simulink library "ammclib_bam_S32K3xx"  (R2016a)
(part 20 of 50)

      |     warning(['Parameter u16NShiftI of ' gcb ' exceeds the fixed-point range.']);
      |   end
      |   f32C1=round(c1f*2^(-u16NShiftI)*2^31);
      |   if f32C1>2^31-1
      |     f32C1=2^31-1;
      |     warning(['Parameter f32C1 of ' gcb ' exceeds the fixed-point range.']);
      |   end
      |   if f32C1<-2^31
      |     f32C1=-2^31;
      |     warning(['Parameter f32C1 of ' gcb ' exceeds the fixed-point range.']);
      |   end
      |   if isnan(f32CC1sc)
      |     if ~strcmp(f32CC1sc_bkup,'0')
      |       set_param(gcb,'f32CC1sc','0');
      |     end
      |   else
      |     tmps=num2str(f32CC1sc);
      |     if ~strcmp(f32CC1sc_bkup,tmps)
      |       set_param(gcb,'f32CC1sc',tmps);
      |     end
      |   end
      |   if isnan(f32CC2sc)
      |     if ~strcmp(f32CC2sc_bkup,'0')
      |       set_param(gcb,'f32CC2sc','0');
      |     end
      |   else
      |     tmps=num2str(f32CC2sc);
      |     if ~strcmp(f32CC2sc_bkup,tmps)
      |       set_param(gcb,'f32CC2sc',tmps);
      |     end
      |   end
      |   if isnan(f32UpperLimit)
      |     if ~strcmp(f32UpperLimit_bkup,'0')
      |       set_param(gcb,'f32UpperLimit','0');
      |     end
      |   else
      |     tmps=num2str(f32UpperLimit);
      |     if ~strcmp(f32UpperLimit_bkup,tmps)
      |       set_param(gcb,'f32UpperLimit',tmps);
      |     end
      |   end
      |   if isnan(f32LowerLimit)
      |     if ~strcmp(f32LowerLimit_bkup,'0')
      |       set_param(gcb,'f32LowerLimit','0');
      |     end
      |   else
      |     tmps=num2str(f32LowerLimit);
      |     if ~strcmp(f32LowerLimit_bkup,tmps)
      |       set_param(gcb,'f32LowerLimit',tmps);
      |     end
      |   end
      |   if isnan(u16NShiftPI)
      |     if ~strcmp(u16NShiftPI_bkup,'0')
      |       set_param(gcb,'u16NShiftPI','0');
      |     end
      |   else
      |     tmps=num2str(u16NShiftPI);
      |     if ~strcmp(u16NShiftPI_bkup,tmps)
      |       set_param(gcb,'u16NShiftPI',tmps);
      |     end
      |   end
      |   if isnan(f32C1)
      |     if ~strcmp(f32C1_bkup,'0')
      |       set_param(gcb,'f32C1','0');
      |     end
      |   else
      |     tmps=num2str(f32C1);
      |     if ~strcmp(f32C1_bkup,tmps)
      |       set_param(gcb,'f32C1',tmps);
      |     end
      |   end
      |   if isnan(u16NShiftI)
      |     if ~strcmp(u16NShiftI_bkup,'0')
      |       set_param(gcb,'u16NShiftI','0');
      |     end
      |   else
      |     tmps=num2str(u16NShiftI);
      |     if ~strcmp(u16NShiftI_bkup,tmps)
      |       set_param(gcb,'u16NShiftI',tmps);
      |     end
      |   end
      | end
      mask Callback if0:
      | autoCalcEn=get_param(gcb,'autoCalcEn');
      | if strcmp(autoCalcEn,'on')
      |   SampleTime=Simulink.data.evalinGlobal(bdroot,get_param(gcb,'SampleTime'));
      |   if (SampleTime==-1)
      |     SampleTime=str2double(get_param(gcb,'SampleTime_1'));
      |   end
      |   f32CC1sc_bkup=get_param(gcb,'f32CC1sc');
      |   f32CC2sc_bkup=get_param(gcb,'f32CC2sc');
      |   f32UpperLimit_bkup=get_param(gcb,'f32UpperLimit');
      |   f32LowerLimit_bkup=get_param(gcb,'f32LowerLimit');
      |   u16NShiftPI_bkup=get_param(gcb,'u16NShiftPI');
      |   f32C1_bkup=get_param(gcb,'f32C1');
      |   u16NShiftI_bkup=get_param(gcb,'u16NShiftI');
      |   intmethod=get_param(gcb,'intmethod');
      |   if0=Simulink.data.evalinGlobal(bdroot,get_param(gcb,'if0'));
      |   iksi=Simulink.data.evalinGlobal(bdroot,get_param(gcb,'iksi'));
      |   mechspeed=Simulink.data.evalinGlobal(bdroot,get_param(gcb,'mechspeed'));
      |   polepairs=Simulink.data.evalinGlobal(bdroot,get_param(gcb,'polepairs'));
      |   if (if0<=0)
      |     warning('Natural frequency f0 must be positive.');
      |   end
      |   if (iksi<=0)
      |     warning('Current loop attenuation must be positive.');
      |   end
      |   if (iksi>1)
      |     warning('Current loop attenuation must not exceed 1.');
      |   end
      |   if (mechspeed<=0)
      |     warning('Max. speed must be positive.');
      |   end
      |   if (polepairs<1)
      |     warning('Number of pole pairs must be a natural number (1, 2, 3, ...).');
      |   end
      |   if (round(polepairs)~=polepairs)
      |     warning('Number of pole pairs must be a natural number (1, 2, 3, ...).');
      |   end
      |   pgain=12.56637061435917*iksi*if0;
      |   igain=39.47841760435743*if0*if0;
      |   if strcmp(intmethod,'Forward Rectangular')
      |     cc1=pgain;
      |     cc2=-pgain+igain*SampleTime;
      |   else
      |     if strcmp(intmethod,'Backward Rectangular')
      |       cc1=pgain+igain*SampleTime;
      |       cc2=-pgain;
      |     else
      |       cc1=pgain+igain*SampleTime*0.5;
      |       cc2=-pgain+igain*SampleTime*0.5;
      |     end
      |   end
      |   wmax=polepairs*mechspeed*0.1047197551196598;
      |   cc1f=cc1*3.141592653589793/wmax;
      |   cc2f=cc2*3.141592653589793/wmax;
      |   u16NShiftPI=ceil(log2(abs(cc1f)));
      |   tmpsh=ceil(log2(abs(cc2f)));
      |   if u16NShiftPI<tmpsh
      |     u16NShiftPI=tmpsh;
      |   end
      |   if u16NShiftPI<0
      |     u16NShiftPI=0;
      |   end
      |   if u16NShiftPI>31
      |     u16NShiftPI=31;
      |     warning(['Parameter u16NShiftPI of ' gcb ' exceeds the fixed-point range.']);
      |   end
      |   f32CC1sc=round(cc1f*2^(-u16NShiftPI)*2^31);
      |   if f32CC1sc>2^31-1
      |     f32CC1sc=2^31-1;
      |     warning(['Parameter f32CC1sc of ' gcb ' exceeds the fixed-point range.']);
      |   end
      |   if f32CC1sc<-2^31
      |     f32CC1sc=-2^31;
      |     warning(['Parameter f32CC1sc of ' gcb ' exceeds the fixed-point range.']);
      |   end
      |   f32CC2sc=round(cc2f*2^(-u16NShiftPI)*2^31);
      |   if f32CC2sc>2^31-1
      |     f32CC2sc=2^31-1;
      |     warning(['Parameter f32CC2sc of ' gcb ' exceeds the fixed-point range.']);
      |   end
      |   if f32CC2sc<-2^31
      |     f32CC2sc=-2^31;
      |     warning(['Parameter f32CC2sc of ' gcb ' exceeds the fixed-point range.']);
      |   end
      |   f32LowerLimit=-2147483648;
      |   f32UpperLimit=2147483647;
      |   c1f=SampleTime*0.5*wmax/3.141592653589793;
      |   u16NShiftI=ceil(log2(abs(c1f)));
      |   if u16NShiftI<0
      |     u16NShiftI=0;
      |   end
      |   if u16NShiftI>31
      |     u16NShiftI=31;
      |     warning(['Parameter u16NShiftI of ' gcb ' exceeds the fixed-point range.']);
      |   end
      |   f32C1=round(c1f*2^(-u16NShiftI)*2^31);
      |   if f32C1>2^31-1
      |     f32C1=2^31-1;
      |     warning(['Parameter f32C1 of ' gcb ' exceeds the fixed-point range.']);
      |   end
      |   if f32C1<-2^31
      |     f32C1=-2^31;
      |     warning(['Parameter f32C1 of ' gcb ' exceeds the fixed-point range.']);
      |   end
      |   if isnan(f32CC1sc)
      |     if ~strcmp(f32CC1sc_bkup,'0')
      |       set_param(gcb,'f32CC1sc','0');
      |     end
      |   else
      |     tmps=num2str(f32CC1sc);
      |     if ~strcmp(f32CC1sc_bkup,tmps)
      |       set_param(gcb,'f32CC1sc',tmps);
      |     end
      |   end
      |   if isnan(f32CC2sc)
      |     if ~strcmp(f32CC2sc_bkup,'0')
      |       set_param(gcb,'f32CC2sc','0');
      |     end
      |   else
      |     tmps=num2str(f32CC2sc);
      |     if ~strcmp(f32CC2sc_bkup,tmps)
      |       set_param(gcb,'f32CC2sc',tmps);
      |     end
      |   end
      |   if isnan(f32UpperLimit)
      |     if ~strcmp(f32UpperLimit_bkup,'0')
      |       set_param(gcb,'f32UpperLimit','0');
      |     end
      |   else
      |     tmps=num2str(f32UpperLimit);
      |     if ~strcmp(f32UpperLimit_bkup,tmps)
      |       set_param(gcb,'f32UpperLimit',tmps);
      |     end
      |   end
      |   if isnan(f32LowerLimit)
      |     if ~strcmp(f32LowerLimit_bkup,'0')
      |       set_param(gcb,'f32LowerLimit','0');
      |     end
      |   else
      |     tmps=num2str(f32LowerLimit);
      |     if ~strcmp(f32LowerLimit_bkup,tmps)
      |       set_param(gcb,'f32LowerLimit',tmps);
      |     end
      |   end
      |   if isnan(u16NShiftPI)
      |     if ~strcmp(u16NShiftPI_bkup,'0')
      |       set_param(gcb,'u16NShiftPI','0');
      |     end
      |   else
      |     tmps=num2str(u16NShiftPI);
      |     if ~strcmp(u16NShiftPI_bkup,tmps)
      |       set_param(gcb,'u16NShiftPI',tmps);
      |     end
      |   end
      |   if isnan(f32C1)
      |     if ~strcmp(f32C1_bkup,'0')
      |       set_param(gcb,'f32C1','0');
      |     end
      |   else
      |     tmps=num2str(f32C1);
      |     if ~strcmp(f32C1_bkup,tmps)
      |       set_param(gcb,'f32C1',tmps);
      |     end
      |   end
      |   if isnan(u16NShiftI)
      |     if ~strcmp(u16NShiftI_bkup,'0')
      |       set_param(gcb,'u16NShiftI','0');
      |     end
      |   else
      |     tmps=num2str(u16NShiftI);
      |     if ~strcmp(u16NShiftI_bkup,tmps)
      |       set_param(gcb,'u16NShiftI',tmps);
      |     end
      |   end
      | end
      mask Callback iksi:
      | autoCalcEn=get_param(gcb,'autoCalcEn');
      | if strcmp(autoCalcEn,'on')
      |   SampleTime=Simulink.data.evalinGlobal(bdroot,get_param(gcb,'SampleTime'));
      |   if (SampleTime==-1)
      |     SampleTime=str2double(get_param(gcb,'SampleTime_1'));
      |   end
      |   f32CC1sc_bkup=get_param(gcb,'f32CC1sc');
      |   f32CC2sc_bkup=get_param(gcb,'f32CC2sc');
      |   f32UpperLimit_bkup=get_param(gcb,'f32UpperLimit');
      |   f32LowerLimit_bkup=get_param(gcb,'f32LowerLimit');
      |   u16NShiftPI_bkup=get_param(gcb,'u16NShiftPI');
      |   f32C1_bkup=get_param(gcb,'f32C1');
      |   u16NShiftI_bkup=get_param(gcb,'u16NShiftI');
      |   intmethod=get_param(gcb,'intmethod');
      |   if0=Simulink.data.evalinGlobal(bdroot,get_param(gcb,'if0'));
      |   iksi=Simulink.data.evalinGlobal(bdroot,get_param(gcb,'iksi'));
      |   mechspeed=Simulink.data.evalinGlobal(bdroot,get_param(gcb,'mechspeed'));
      |   polepairs=Simulink.data.evalinGlobal(bdroot,get_param(gcb,'polepairs'));
      |   if (if0<=0)
      |     warning('Natural frequency f0 must be positive.');
      |   end
      |   if (iksi<=0)
      |     warning('Current loop attenuation must be positive.');
      |   end
      |   if (iksi>1)
      |     warning('Current loop attenuation must not exceed 1.');
      |   end
      |   if (mechspeed<=0)
      |     warning('Max. speed must be positive.');
      |   end
      |   if (polepairs<1)
      |     warning('Number of pole pairs must be a natural number (1, 2, 3, ...).');
      |   end
      |   if (round(polepairs)~=polepairs)
      |     warning('Number of pole pairs must be a natural number (1, 2, 3, ...).');
      |   end
      |   pgain=12.56637061435917*iksi*if0;
      |   igain=39.47841760435743*if0*if0;
      |   if strcmp(intmethod,'Forward Rectangular')
      |     cc1=pgain;
      |     cc2=-pgain+igain*SampleTime;
      |   else
      |     if strcmp(intmethod,'Backward Rectangular')
      |       cc1=pgain+igain*SampleTime;
      |       cc2=-pgain;
      |     else
      |       cc1=pgain+igain*SampleTime*0.5;
      |       cc2=-pgain+igain*SampleTime*0.5;
      |     end
      |   end
      |   wmax=polepairs*mechspeed*0.1047197551196598;
      |   cc1f=cc1*3.141592653589793/wmax;
      |   cc2f=cc2*3.141592653589793/wmax;
      |   u16NShiftPI=ceil(log2(abs(cc1f)));
      |   tmpsh=ceil(log2(abs(cc2f)));
      |   if u16NShiftPI<tmpsh
      |     u16NShiftPI=tmpsh;
      |   end
      |   if u16NShiftPI<0
      |     u16NShiftPI=0;
      |   end
      |   if u16NShiftPI>31
      |     u16NShiftPI=31;
      |     warning(['Parameter u16NShiftPI of ' gcb ' exceeds the fixed-point range.']);
      |   end
      |   f32CC1sc=round(cc1f*2^(-u16NShiftPI)*2^31);
      |   if f32CC1sc>2^31-1
      |     f32CC1sc=2^31-1;
      |     warning(['Parameter f32CC1sc of ' gcb ' exceeds the fixed-point range.']);
      |   end
      |   if f32CC1sc<-2^31
      |     f32CC1sc=-2^31;
      |     warning(['Parameter f32CC1sc of ' gcb ' exceeds the fixed-point range.']);
      |   end
      |   f32CC2sc=round(cc2f*2^(-u16NShiftPI)*2^31);
      |   if f32CC2sc>2^31-1
      |     f32CC2sc=2^31-1;
      |     warning(['Parameter f32CC2sc of ' gcb ' exceeds the fixed-point range.']);
      |   end
      |   if f32CC2sc<-2^31
      |     f32CC2sc=-2^31;
      |     warning(['Parameter f32CC2sc of ' gcb ' exceeds the fixed-point range.']);
      |   end
      |   f32LowerLimit=-2147483648;
      |   f32UpperLimit=2147483647;
      |   c1f=SampleTime*0.5*wmax/3.141592653589793;
      |   u16NShiftI=ceil(log2(abs(c1f)));
      |   if u16NShiftI<0
      |     u16NShiftI=0;
      |   end
      |   if u16NShiftI>31
      |     u16NShiftI=31;
      |     warning(['Parameter u16NShiftI of ' gcb ' exceeds the fixed-point range.']);
      |   end
      |   f32C1=round(c1f*2^(-u16NShiftI)*2^31);
      |   if f32C1>2^31-1
      |     f32C1=2^31-1;
      |     warning(['Parameter f32C1 of ' gcb ' exceeds the fixed-point range.']);
      |   end
      |   if f32C1<-2^31
      |     f32C1=-2^31;
      |     warning(['Parameter f32C1 of ' gcb ' exceeds the fixed-point range.']);
      |   end
      |   if isnan(f32CC1sc)
      |     if ~strcmp(f32CC1sc_bkup,'0')
      |       set_param(gcb,'f32CC1sc','0');
      |     end
      |   else
      |     tmps=num2str(f32CC1sc);
      |     if ~strcmp(f32CC1sc_bkup,tmps)
      |       set_param(gcb,'f32CC1sc',tmps);
      |     end
      |   end
      |   if isnan(f32CC2sc)
      |     if ~strcmp(f32CC2sc_bkup,'0')
      |       set_param(gcb,'f32CC2sc','0');
      |     end
      |   else
      |     tmps=num2str(f32CC2sc);
      |     if ~strcmp(f32CC2sc_bkup,tmps)
      |       set_param(gcb,'f32CC2sc',tmps);
      |     end
      |   end
      |   if isnan(f32UpperLimit)
      |     if ~strcmp(f32UpperLimit_bkup,'0')
      |       set_param(gcb,'f32UpperLimit','0');
      |     end
      |   else
      |     tmps=num2str(f32UpperLimit);
      |     if ~strcmp(f32UpperLimit_bkup,tmps)
      |       set_param(gcb,'f32UpperLimit',tmps);
      |     end
      |   end
      |   if isnan(f32LowerLimit)
      |     if ~strcmp(f32LowerLimit_bkup,'0')
      |       set_param(gcb,'f32LowerLimit','0');
      |     end
      |   else
      |     tmps=num2str(f32LowerLimit);
      |     if ~strcmp(f32LowerLimit_bkup,tmps)
      |       set_param(gcb,'f32LowerLimit',tmps);
      |     end
      |   end
      |   if isnan(u16NShiftPI)
      |     if ~strcmp(u16NShiftPI_bkup,'0')
      |       set_param(gcb,'u16NShiftPI','0');
      |     end
      |   else
      |     tmps=num2str(u16NShiftPI);
      |     if ~strcmp(u16NShiftPI_bkup,tmps)
      |       set_param(gcb,'u16NShiftPI',tmps);
      |     end
      |   end
      |   if isnan(f32C1)
      |     if ~strcmp(f32C1_bkup,'0')
      |       set_param(gcb,'f32C1','0');
      |     end
      |   else
      |     tmps=num2str(f32C1);
      |     if ~strcmp(f32C1_bkup,tmps)
      |       set_param(gcb,'f32C1',tmps);
      |     end
      |   end
      |   if isnan(u16NShiftI)
      |     if ~strcmp(u16NShiftI_bkup,'0')
      |       set_param(gcb,'u16NShiftI','0');
      |     end
      |   else
      |     tmps=num2str(u16NShiftI);
      |     if ~strcmp(u16NShiftI_bkup,tmps)
      |       set_param(gcb,'u16NShiftI',tmps);
      |     end
      |   end
      | end
      mask Callback mechspeed:
      | autoCalcEn=get_param(gcb,'autoCalcEn');
      | if strcmp(autoCalcEn,'on')
      |   SampleTime=Simulink.data.evalinGlobal(bdroot,get_param(gcb,'SampleTime'));
      |   if (SampleTime==-1)
      |     SampleTime=str2double(get_param(gcb,'SampleTime_1'));
      |   end
      |   f32CC1sc_bkup=get_param(gcb,'f32CC1sc');
      |   f32CC2sc_bkup=get_param(gcb,'f32CC2sc');
      |   f32UpperLimit_bkup=get_param(gcb,'f32UpperLimit');
      |   f32LowerLimit_bkup=get_param(gcb,'f32LowerLimit');
      |   u16NShiftPI_bkup=get_param(gcb,'u16NShiftPI');
      |   f32C1_bkup=get_param(gcb,'f32C1');
      |   u16NShiftI_bkup=get_param(gcb,'u16NShiftI');
      |   intmethod=get_param(gcb,'intmethod');
      |   if0=Simulink.data.evalinGlobal(bdroot,get_param(gcb,'if0'));
      |   iksi=Simulink.data.evalinGlobal(bdroot,get_param(gcb,'iksi'));
      |   mechspeed=Simulink.data.evalinGlobal(bdroot,get_param(gcb,'mechspeed'));
      |   polepairs=Simulink.data.evalinGlobal(bdroot,get_param(gcb,'polepairs'));
      |   if (if0<=0)
      |     warning('Natural frequency f0 must be positive.');
      |   end
      |   if (iksi<=0)
      |     warning('Current loop attenuation must be positive.');
      |   end
      |   if (iksi>1)
      |     warning('Current loop attenuation must not exceed 1.');
      |   end
      |   if (mechspeed<=0)
      |     warning('Max. speed must be positive.');
      |   end
      |   if (polepairs<1)
      |     warning('Number of pole pairs must be a natural number (1, 2, 3, ...).');
      |   end
      |   if (round(polepairs)~=polepairs)
      |     warning('Number of pole pairs must be a natural number (1, 2, 3, ...).');
      |   end
      |   pgain=12.56637061435917*iksi*if0;
      |   igain=39.47841760435743*if0*if0;
      |   if strcmp(intmethod,'Forward Rectangular')
      |     cc1=pgain;
      |     cc2=-pgain+igain*SampleTime;
      |   else
      |     if strcmp(intmethod,'Backward Rectangular')
      |       cc1=pgain+igain*SampleTime;
      |       cc2=-pgain;
      |     else
      |       cc1=pgain+igain*SampleTime*0.5;
      |       cc2=-pgain+igain*SampleTime*0.5;
      |     end
      |   end
      |   wmax=polepairs*mechspeed*0.1047197551196598;
      |   cc1f=cc1*3.141592653589793/wmax;
      |   cc2f=cc2*3.141592653589793/wmax;
      |   u16NShiftPI=ceil(log2(abs(cc1f)));
      |   tmpsh=ceil(log2(abs(cc2f)));
      |   if u16NShiftPI<tmpsh
      |     u16NShiftPI=tmpsh;
      |   end
      |   if u16NShiftPI<0
      |     u16NShiftPI=0;
      |   end
      |   if u16NShiftPI>31
      |     u16NShiftPI=31;
      |     warning(['Parameter u16NShiftPI of ' gcb ' exceeds the fixed-point range.']);
      |   end
      |   f32CC1sc=round(cc1f*2^(-u16NShiftPI)*2^31);
      |   if f32CC1sc>2^31-1
      |     f32CC1sc=2^31-1;
      |     warning(['Parameter f32CC1sc of ' gcb ' exceeds the fixed-point range.']);
      |   end
      |   if f32CC1sc<-2^31
      |     f32CC1sc=-2^31;
      |     warning(['Parameter f32CC1sc of ' gcb ' exceeds the fixed-point range.']);
      |   end
      |   f32CC2sc=round(cc2f*2^(-u16NShiftPI)*2^31);
      |   if f32CC2sc>2^31-1
      |     f32CC2sc=2^31-1;
      |     warning(['Parameter f32CC2sc of ' gcb ' exceeds the fixed-point range.']);
      |   end
      |   if f32CC2sc<-2^31
      |     f32CC2sc=-2^31;
      |     warning(['Parameter f32CC2sc of ' gcb ' exceeds the fixed-point range.']);
      |   end
      |   f32LowerLimit=-2147483648;
      |   f32UpperLimit=2147483647;
      |   c1f=SampleTime*0.5*wmax/3.141592653589793;
      |   u16NShiftI=ceil(log2(abs(c1f)));
      |   if u16NShiftI<0
      |     u16NShiftI=0;
      |   end
      |   if u16NShiftI>31
      |     u16NShiftI=31;
      |     warning(['Parameter u16NShiftI of ' gcb ' exceeds the fixed-point range.']);
      |   end
      |   f32C1=round(c1f*2^(-u16NShiftI)*2^31);
      |   if f32C1>2^31-1
      |     f32C1=2^31-1;
      |     warning(['Parameter f32C1 of ' gcb ' exceeds the fixed-point range.']);
      |   end
      |   if f32C1<-2^31
      |     f32C1=-2^31;
      |     warning(['Parameter f32C1 of ' gcb ' exceeds the fixed-point range.']);
      |   end
      |   if isnan(f32CC1sc)
      |     if ~strcmp(f32CC1sc_bkup,'0')
      |       set_param(gcb,'f32CC1sc','0');
      |     end
      |   else
      |     tmps=num2str(f32CC1sc);
      |     if ~strcmp(f32CC1sc_bkup,tmps)
      |       set_param(gcb,'f32CC1sc',tmps);
      |     end
      |   end
      |   if isnan(f32CC2sc)
      |     if ~strcmp(f32CC2sc_bkup,'0')
      |       set_param(gcb,'f32CC2sc','0');
      |     end
      |   else
      |     tmps=num2str(f32CC2sc);
      |     if ~strcmp(f32CC2sc_bkup,tmps)
      |       set_param(gcb,'f32CC2sc',tmps);
      |     end
      |   end
      |   if isnan(f32UpperLimit)
      |     if ~strcmp(f32UpperLimit_bkup,'0')
      |       set_param(gcb,'f32UpperLimit','0');
      |     end
      |   else
      |     tmps=num2str(f32UpperLimit);
      |     if ~strcmp(f32UpperLimit_bkup,tmps)
      |       set_param(gcb,'f32UpperLimit',tmps);
      |     end
      |   end
      |   if isnan(f32LowerLimit)
      |     if ~strcmp(f32LowerLimit_bkup,'0')
      |       set_param(gcb,'f32LowerLimit','0');
      |     end
      |   else
      |     tmps=num2str(f32LowerLimit);
      |     if ~strcmp(f32LowerLimit_bkup,tmps)
      |       set_param(gcb,'f32LowerLimit',tmps);
      |     end
      |   end
      |   if isnan(u16NShiftPI)
      |     if ~strcmp(u16NShiftPI_bkup,'0')
      |       set_param(gcb,'u16NShiftPI','0');
      |     end
      |   else
      |     tmps=num2str(u16NShiftPI);
      |     if ~strcmp(u16NShiftPI_bkup,tmps)
      |       set_param(gcb,'u16NShiftPI',tmps);
      |     end
      |   end
      |   if isnan(f32C1)
      |     if ~strcmp(f32C1_bkup,'0')
      |       set_param(gcb,'f32C1','0');
      |     end
      |   else
      |     tmps=num2str(f32C1);
      |     if ~strcmp(f32C1_bkup,tmps)
      |       set_param(gcb,'f32C1',tmps);
      |     end
      |   end
      |   if isnan(u16NShiftI)
      |     if ~strcmp(u16NShiftI_bkup,'0')
      |       set_param(gcb,'u16NShiftI','0');
      |     end
      |   else
      |     tmps=num2str(u16NShiftI);
      |     if ~strcmp(u16NShiftI_bkup,tmps)
      |       set_param(gcb,'u16NShiftI',tmps);
      |     end
      |   end
      | end
      mask Callback polepairs:
      | autoCalcEn=get_param(gcb,'autoCalcEn');
      | if strcmp(autoCalcEn,'on')
      |   SampleTime=Simulink.data.evalinGlobal(bdroot,get_param(gcb,'SampleTime'));
      |   if (SampleTime==-1)
      |     SampleTime=str2double(get_param(gcb,'SampleTime_1'));
      |   end
      |   f32CC1sc_bkup=get_param(gcb,'f32CC1sc');
      |   f32CC2sc_bkup=get_param(gcb,'f32CC2sc');
      |   f32UpperLimit_bkup=get_param(gcb,'f32UpperLimit');
      |   f32LowerLimit_bkup=get_param(gcb,'f32LowerLimit');
      |   u16NShiftPI_bkup=get_param(gcb,'u16NShiftPI');
      |   f32C1_bkup=get_param(gcb,'f32C1');
      |   u16NShiftI_bkup=get_param(gcb,'u16NShiftI');
      |   intmethod=get_param(gcb,'intmethod');
      |   if0=Simulink.data.evalinGlobal(bdroot,get_param(gcb,'if0'));
      |   iksi=Simulink.data.evalinGlobal(bdroot,get_param(gcb,'iksi'));
      |   mechspeed=Simulink.data.evalinGlobal(bdroot,get_param(gcb,'mechspeed'));
      |   polepairs=Simulink.data.evalinGlobal(bdroot,get_param(gcb,'polepairs'));
      |   if (if0<=0)
      |     warning('Natural frequency f0 must be positive.');
      |   end
      |   if (iksi<=0)
      |     warning('Current loop attenuation must be positive.');
      |   end
      |   if (iksi>1)
      |     warning('Current loop attenuation must not exceed 1.');
      |   end
      |   if (mechspeed<=0)
      |     warning('Max. speed must be positive.');
      |   end
      |   if (polepairs<1)
      |     warning('Number of pole pairs must be a natural number (1, 2, 3, ...).');
      |   end
      |   if (round(polepairs)~=polepairs)
      |     warning('Number of pole pairs must be a natural number (1, 2, 3, ...).');
      |   end
      |   pgain=12.56637061435917*iksi*if0;
      |   igain=39.47841760435743*if0*if0;
      |   if strcmp(intmethod,'Forward Rectangular')
      |     cc1=pgain;
      |     cc2=-pgain+igain*SampleTime;
      |   else
      |     if strcmp(intmethod,'Backward Rectangular')
      |       cc1=pgain+igain*SampleTime;
      |       cc2=-pgain;
      |     else
      |       cc1=pgain+igain*SampleTime*0.5;
      |       cc2=-pgain+igain*SampleTime*0.5;
      |     end
      |   end
      |   wmax=polepairs*mechspeed*0.1047197551196598;
      |   cc1f=cc1*3.141592653589793/wmax;
      |   cc2f=cc2*3.141592653589793/wmax;
      |   u16NShiftPI=ceil(log2(abs(cc1f)));
      |   tmpsh=ceil(log2(abs(cc2f)));
      |   if u16NShiftPI<tmpsh
      |     u16NShiftPI=tmpsh;
      |   end
      |   if u16NShiftPI<0
      |     u16NShiftPI=0;
      |   end
      |   if u16NShiftPI>31
      |     u16NShiftPI=31;
      |     warning(['Parameter u16NShiftPI of ' gcb ' exceeds the fixed-point range.']);
      |   end
      |   f32CC1sc=round(cc1f*2^(-u16NShiftPI)*2^31);
      |   if f32CC1sc>2^31-1
      |     f32CC1sc=2^31-1;
      |     warning(['Parameter f32CC1sc of ' gcb ' exceeds the fixed-point range.']);
      |   end
      |   if f32CC1sc<-2^31
      |     f32CC1sc=-2^31;
      |     warning(['Parameter f32CC1sc of ' gcb ' exceeds the fixed-point range.']);
      |   end
      |   f32CC2sc=round(cc2f*2^(-u16NShiftPI)*2^31);
      |   if f32CC2sc>2^31-1
      |     f32CC2sc=2^31-1;
      |     warning(['Parameter f32CC2sc of ' gcb ' exceeds the fixed-point range.']);
      |   end
      |   if f32CC2sc<-2^31
      |     f32CC2sc=-2^31;
      |     warning(['Parameter f32CC2sc of ' gcb ' exceeds the fixed-point range.']);
      |   end
      |   f32LowerLimit=-2147483648;
      |   f32UpperLimit=2147483647;
      |   c1f=SampleTime*0.5*wmax/3.141592653589793;
      |   u16NShiftI=ceil(log2(abs(c1f)));
      |   if u16NShiftI<0
      |     u16NShiftI=0;
      |   end
      |   if u16NShiftI>31
      |     u16NShiftI=31;
      |     warning(['Parameter u16NShiftI of ' gcb ' exceeds the fixed-point range.']);
      |   end
      |   f32C1=round(c1f*2^(-u16NShiftI)*2^31);
      |   if f32C1>2^31-1
      |     f32C1=2^31-1;
      |     warning(['Parameter f32C1 of ' gcb ' exceeds the fixed-point range.']);
      |   end
      |   if f32C1<-2^31
      |     f32C1=-2^31;
      |     warning(['Parameter f32C1 of ' gcb ' exceeds the fixed-point range.']);
      |   end
      |   if isnan(f32CC1sc)
      |     if ~strcmp(f32CC1sc_bkup,'0')
      |       set_param(gcb,'f32CC1sc','0');
      |     end
      |   else
      |     tmps=num2str(f32CC1sc);
      |     if ~strcmp(f32CC1sc_bkup,tmps)
      |       set_param(gcb,'f32CC1sc',tmps);
      |     end
      |   end
      |   if isnan(f32CC2sc)
      |     if ~strcmp(f32CC2sc_bkup,'0')
      |       set_param(gcb,'f32CC2sc','0');
      |     end
      |   else
      |     tmps=num2str(f32CC2sc);
      |     if ~strcmp(f32CC2sc_bkup,tmps)
      |       set_param(gcb,'f32CC2sc',tmps);
      |     end
      |   end
      |   if isnan(f32UpperLimit)
      |     if ~strcmp(f32UpperLimit_bkup,'0')
      |       set_param(gcb,'f32UpperLimit','0');
      |     end
      |   else
      |     tmps=num2str(f32UpperLimit);
      |     if ~strcmp(f32UpperLimit_bkup,tmps)
      |       set_param(gcb,'f32UpperLimit',tmps);
      |     end
      |   end
      |   if isnan(f32LowerLimit)
      |     if ~strcmp(f32LowerLimit_bkup,'0')
      |       set_param(gcb,'f32LowerLimit','0');
      |     end
      |   else
      |     tmps=num2str(f32LowerLimit);
      |     if ~strcmp(f32LowerLimit_bkup,tmps)
      |       set_param(gcb,'f32LowerLimit',tmps);
      |     end
      |   end
      |   if isnan(u16NShiftPI)
      |     if ~strcmp(u16NShiftPI_bkup,'0')
      |       set_param(gcb,'u16NShiftPI','0');
      |     end
      |   else
      |     tmps=num2str(u16NShiftPI);
      |     if ~strcmp(u16NShiftPI_bkup,tmps)
      |       set_param(gcb,'u16NShiftPI',tmps);
      |     end
      |   end
      |   if isnan(f32C1)
      |     if ~strcmp(f32C1_bkup,'0')
      |       set_param(gcb,'f32C1','0');
      |     end
      |   else
      |     tmps=num2str(f32C1);
      |     if ~strcmp(f32C1_bkup,tmps)
      |       set_param(gcb,'f32C1',tmps);
      |     end
      |   end
      |   if isnan(u16NShiftI)
      |     if ~strcmp(u16NShiftI_bkup,'0')
      |       set_param(gcb,'u16NShiftI','0');
      |     end
      |   else
      |     tmps=num2str(u16NShiftI);
      |     if ~strcmp(u16NShiftI_bkup,tmps)
      |       set_param(gcb,'u16NShiftI',tmps);
      |     end
      |   end
      | end
      mask Callback autoCalcEn:
      | maskStr=get_param(gcb,'showStates');
      | if strcmp(maskStr,'Hide (faster execution)')
      |   p=Simulink.Mask.get(gcb);
      |   autoCalcEn=get_param(gcb,'autoCalcEn');
      |   hintText=p.getDialogControl('timeHint');
      |   if strcmp(autoCalcEn,'on')
      |     param=p.getParameter('polepairs');
      |     if strcmp(param.Enabled,'off')
      |       SampleTime=Simulink.data.evalinGlobal(bdroot,get_param(gcb,'SampleTime'));
      |       if SampleTime==-1
      |         SampleTime=str2double(get_param(gcb,'SampleTime_1'));
      |         if isnan(SampleTime)
      |           hintText.Prompt=['Note: Implementation parameters cannot be calculated yet because the block''s inherited sample time is unknown. Simulink will update the sample time when you run the simulation.'];
      |         else
      |           hintText.Prompt=['Caution: Implementation parameters depend on inherited sample time. Make sure that the sample time of the block''s inputs corresponds to the sampling period in the target application.'];
      |         end
      |       else
      |         hintText.Prompt='Caution: Implementation parameters depend on the sample time. Make sure that the simulation time step corresponds to the sampling period in the target application.';
      |       end
      |       p=Simulink.Mask.get(gcb);
      |       param=p.getParameter('intmethod');
      |       param.set('Enabled','on');
      |       param=p.getParameter('if0');
      |       param.set('Enabled','on');
      |       param=p.getParameter('iksi');
      |       param.set('Enabled','on');
      |       param=p.getParameter('mechspeed');
      |       param.set('Enabled','on');
      |       param=p.getParameter('polepairs');
      |       param.set('Enabled','on');
      |     else
      |       SampleTime=Simulink.data.evalinGlobal(bdroot,get_param(gcb,'SampleTime'));
      |       if SampleTime==-1
      |         SampleTime=str2double(get_param(gcb,'SampleTime_1'));
      |       end
      |     end
      |     f32CC1sc_bkup=get_param(gcb,'f32CC1sc');
      |     f32CC2sc_bkup=get_param(gcb,'f32CC2sc');
      |     f32UpperLimit_bkup=get_param(gcb,'f32UpperLimit');
      |     f32LowerLimit_bkup=get_param(gcb,'f32LowerLimit');
      |     u16NShiftPI_bkup=get_param(gcb,'u16NShiftPI');
      |     f32C1_bkup=get_param(gcb,'f32C1');
      |     u16NShiftI_bkup=get_param(gcb,'u16NShiftI');
      |     intmethod=get_param(gcb,'intmethod');
      |     if0=Simulink.data.evalinGlobal(bdroot,get_param(gcb,'if0'));
      |     iksi=Simulink.data.evalinGlobal(bdroot,get_param(gcb,'iksi'));
      |     mechspeed=Simulink.data.evalinGlobal(bdroot,get_param(gcb,'mechspeed'));
      |     polepairs=Simulink.data.evalinGlobal(bdroot,get_param(gcb,'polepairs'));
      |     if (if0<=0)
      |       warning('Natural frequency f0 must be positive.');
      |     end
      |     if (iksi<=0)
      |       warning('Current loop attenuation must be positive.');
      |     end
      |     if (iksi>1)
      |       warning('Current loop attenuation must not exceed 1.');
      |     end
      |     if (mechspeed<=0)
      |       warning('Max. speed must be positive.');
      |     end
      |     if (polepairs<1)
      |       warning('Number of pole pairs must be a natural number (1, 2, 3, ...).');
      |     end
      |     if (round(polepairs)~=polepairs)
      |       warning('Number of pole pairs must be a natural number (1, 2, 3, ...).');
      |     end
      |     pgain=12.56637061435917*iksi*if0;
      |     igain=39.47841760435743*if0*if0;
      |     if strcmp(intmethod,'Forward Rectangular')
      |       cc1=pgain;
      |       cc2=-pgain+igain*SampleTime;
      |     else
      |       if strcmp(intmethod,'Backward Rectangular')
      |         cc1=pgain+igain*SampleTime;
      |         cc2=-pgain;
      |       else
      |         cc1=pgain+igain*SampleTime*0.5;
      |         cc2=-pgain+igain*SampleTime*0.5;
      |       end
      |     end
      |     wmax=polepairs*mechspeed*0.1047197551196598;
      |     cc1f=cc1*3.141592653589793/wmax;
      |     cc2f=cc2*3.141592653589793/wmax;
      |     u16NShiftPI=ceil(log2(abs(cc1f)));
      |     tmpsh=ceil(log2(abs(cc2f)));
      |     if u16NShiftPI<tmpsh
      |       u16NShiftPI=tmpsh;
      |     end
      |     if u16NShiftPI<0
      |       u16NShiftPI=0;
      |     end
      |     if u16NShiftPI>31
      |       u16NShiftPI=31;
      |       warning(['Parameter u16NShiftPI of ' gcb ' exceeds the fixed-point range.']);
      |     end
      |     f32CC1sc=round(cc1f*2^(-u16NShiftPI)*2^31);
      |     if f32CC1sc>2^31-1
      |       f32CC1sc=2^31-1;
      |       warning(['Parameter f32CC1sc of ' gcb ' exceeds the fixed-point range.']);
      |     end
      |     if f32CC1sc<-2^31
      |       f32CC1sc=-2^31;
      |       warning(['Parameter f32CC1sc of ' gcb ' exceeds the fixed-point range.']);
      |     end
      |     f32CC2sc=round(cc2f*2^(-u16NShiftPI)*2^31);
      |     if f32CC2sc>2^31-1
      |       f32CC2sc=2^31-1;
      |       warning(['Parameter f32CC2sc of ' gcb ' exceeds the fixed-point range.']);
      |     end
      |     if f32CC2sc<-2^31
      |       f32CC2sc=-2^31;
      |       warning(['Parameter f32CC2sc of ' gcb ' exceeds the fixed-point range.']);
      |     end
      |     f32LowerLimit=-2147483648;
      |     f32UpperLimit=2147483647;
      |     c1f=SampleTime*0.5*wmax/3.141592653589793;
      |     u16NShiftI=ceil(log2(abs(c1f)));
      |     if u16NShiftI<0
      |       u16NShiftI=0;
      |     end
      |     if u16NShiftI>31
      |       u16NShiftI=31;
      |       warning(['Parameter u16NShiftI of ' gcb ' exceeds the fixed-point range.']);
      |     end
      |     f32C1=round(c1f*2^(-u16NShiftI)*2^31);
      |     if f32C1>2^31-1
      |       f32C1=2^31-1;
      |       warning(['Parameter f32C1 of ' gcb ' exceeds the fixed-point range.']);
      |     end
      |     if f32C1<-2^31
      |       f32C1=-2^31;
      |       warning(['Parameter f32C1 of ' gcb ' exceeds the fixed-point range.']);
      |     end
      |     if isnan(f32CC1sc)
      |       if ~strcmp(f32CC1sc_bkup,'0')
      |         set_param(gcb,'f32CC1sc','0');
      |       end
      |     else
      |       tmps=num2str(f32CC1sc);
      |       if ~strcmp(f32CC1sc_bkup,tmps)
      |         set_param(gcb,'f32CC1sc',tmps);
      |       end
      |     end
      |     if isnan(f32CC2sc)
      |       if ~strcmp(f32CC2sc_bkup,'0')
      |         set_param(gcb,'f32CC2sc','0');
      |       end
      |     else
      |       tmps=num2str(f32CC2sc);
      |       if ~strcmp(f32CC2sc_bkup,tmps)
      |         set_param(gcb,'f32CC2sc',tmps);
      |       end
      |     end
      |     if isnan(f32UpperLimit)
      |       if ~strcmp(f32UpperLimit_bkup,'0')
      |         set_param(gcb,'f32UpperLimit','0');
      |       end
      |     else
      |       tmps=num2str(f32UpperLimit);
      |       if ~strcmp(f32UpperLimit_bkup,tmps)
      |         set_param(gcb,'f32UpperLimit',tmps);
      |       end
      |     end
      |     if isnan(f32LowerLimit)
      |       if ~strcmp(f32LowerLimit_bkup,'0')
      |         set_param(gcb,'f32LowerLimit','0');
      |       end
      |     else
      |       tmps=num2str(f32LowerLimit);
      |       if ~strcmp(f32LowerLimit_bkup,tmps)
      |         set_param(gcb,'f32LowerLimit',tmps);
      |       end
      |     end
      |     if isnan(u16NShiftPI)
      |       if ~strcmp(u16NShiftPI_bkup,'0')
      |         set_param(gcb,'u16NShiftPI','0');
      |       end
      |     else
      |       tmps=num2str(u16NShiftPI);
      |       if ~strcmp(u16NShiftPI_bkup,tmps)
      |         set_param(gcb,'u16NShiftPI',tmps);
      |       end
      |     end
      |     if isnan(f32C1)
      |       if ~strcmp(f32C1_bkup,'0')
      |         set_param(gcb,'f32C1','0');
      |       end
      |     else
      |       tmps=num2str(f32C1);
      |       if ~strcmp(f32C1_bkup,tmps)
      |         set_param(gcb,'f32C1',tmps);
      |       end
      |     end
      |     if isnan(u16NShiftI)
      |       if ~strcmp(u16NShiftI_bkup,'0')
      |         set_param(gcb,'u16NShiftI','0');
      |       end
      |     else
      |       tmps=num2str(u16NShiftI);
      |       if ~strcmp(u16NShiftI_bkup,tmps)
      |         set_param(gcb,'u16NShiftI',tmps);
      |       end
      |     end
      |   else
      |     param=p.getParameter('polepairs');
      |     if strcmp(param.Enabled,'on')
      |       hintText.Prompt='Caution: Implementation parameters are fixed.';
      |       p=Simulink.Mask.get(gcb);
      |       param=p.getParameter('intmethod');
      |       param.set('Enabled','off');
      |       param=p.getParameter('if0');
      |       param.set('Enabled','off');
      |       param=p.getParameter('iksi');
      |       param.set('Enabled','off');
      |       param=p.getParameter('mechspeed');
      |       param.set('Enabled','off');
      |       param=p.getParameter('polepairs');
      |       param.set('Enabled','off');
      |     end
      |   end
      | end
      mask DialogControl CompBut Prompt: Recalculate sample times
      mask DialogControl CompBut Tooltip: Simulink updates the sample times of all blocks when the simulation is run. This button will update the sample times now.
      mask DialogControl CompBut Callback:
      | btn=questdlg('This will apply all changes in all open dialog boxes and update the schematic. Do you want to proceed?','Apply all changes','Continue','Cancel','Continue');
      | if strcmp(btn,'Continue')
      |   dlgs=DAStudio.ToolRoot.getOpenDialogs;
      |   for i=1:length(dlgs)
      |     dlgs(i).apply;
      |   end
      |   try
      |     SampleTime_1=str2double(get_param(gcb,'SampleTime_1'));
      |     ts=Simulink.Block.getSampleTimes(gcb);
      |     ts=ts(1).Value(1);
      |     if (SampleTime_1 ~= ts)
      |       SampleTime_1=ts;
      |       set_param(gcb,'SampleTime_1',num2str(ts));
      |       autoCalcEn=get_param(gcb,'autoCalcEn');
      |       if strcmp(autoCalcEn,'on')
      |         SampleTime=Simulink.data.evalinGlobal(bdroot,get_param(gcb,'SampleTime'));
      |         p=Simulink.Mask.get(gcb);
      |         hintText=p.getDialogControl('timeHint');
      |         if SampleTime==-1
      |           SampleTime=SampleTime_1;
      |           hintText.Prompt='Caution: Implementation parameters depend on inherited sample time. Make sure that the sample time of the block''s inputs corresponds to the sampling period in the target application.';
      |         else
      |           hintText.Prompt='Caution: Implementation parameters depend on the sample time. Make sure that the simulation time step corresponds to the sampling period in the target application.';
      |         end
      |         f32CC1sc_bkup=get_param(gcb,'f32CC1sc');
      |         f32CC2sc_bkup=get_param(gcb,'f32CC2sc');
      |         f32UpperLimit_bkup=get_param(gcb,'f32UpperLimit');
      |         f32LowerLimit_bkup=get_param(gcb,'f32LowerLimit');
      |         u16NShiftPI_bkup=get_param(gcb,'u16NShiftPI');
      |         f32C1_bkup=get_param(gcb,'f32C1');
      |         u16NShiftI_bkup=get_param(gcb,'u16NShiftI');
      |         intmethod=get_param(gcb,'intmethod');
      |         if0=Simulink.data.evalinGlobal(bdroot,get_param(gcb,'if0'));
      |         iksi=Simulink.data.evalinGlobal(bdroot,get_param(gcb,'iksi'));
      |         mechspeed=Simulink.data.evalinGlobal(bdroot,get_param(gcb,'mechspeed'));
      |         polepairs=Simulink.data.evalinGlobal(bdroot,get_param(gcb,'polepairs'));
      |         if (if0<=0)
      |           warning('Natural frequency f0 must be positive.');
      |         end
      |         if (iksi<=0)
      |           warning('Current loop attenuation must be positive.');
      |         end
      |         if (iksi>1)
      |           warning('Current loop attenuation must not exceed 1.');
      |         end
      |         if (mechspeed<=0)
      |           warning('Max. speed must be positive.');
      |         end
      |         if (polepairs<1)
      |           warning('Number of pole pairs must be a natural number (1, 2, 3, ...).');
      |         end
      |         if (round(polepairs)~=polepairs)
      |           warning('Number of pole pairs must be a natural number (1, 2, 3, ...).');
      |         end
      |         pgain=12.56637061435917*iksi*if0;
      |         igain=39.47841760435743*if0*if0;
      |         if strcmp(intmethod,'Forward Rectangular')
      |           cc1=pgain;
      |           cc2=-pgain+igain*SampleTime;
      |         else
      |           if strcmp(intmethod,'Backward Rectangular')
      |             cc1=pgain+igain*SampleTime;
      |             cc2=-pgain;
      |           else
      |             cc1=pgain+igain*SampleTime*0.5;
      |             cc2=-pgain+igain*SampleTime*0.5;
      |           end
      |         end
      |         wmax=polepairs*mechspeed*0.1047197551196598;
      |         cc1f=cc1*3.141592653589793/wmax;
      |         cc2f=cc2*3.141592653589793/wmax;
      |         u16NShiftPI=ceil(log2(abs(cc1f)));
      |         tmpsh=ceil(log2(abs(cc2f)));
      |         if u16NShiftPI<tmpsh
      |           u16NShiftPI=tmpsh;
      |         end
      |         if u16NShiftPI<0
      |           u16NShiftPI=0;
      |         end
      |         if u16NShiftPI>31
      |           u16NShiftPI=31;
      |           warning(['Parameter u16NShiftPI of ' gcb ' exceeds the fixed-point range.']);
      |         end
      |         f32CC1sc=round(cc1f*2^(-u16NShiftPI)*2^31);
      |         if f32CC1sc>2^31-1
      |           f32CC1sc=2^31-1;
      |           warning(['Parameter f32CC1sc of ' gcb ' exceeds the fixed-point range.']);
      |         end
      |         if f32CC1sc<-2^31
      |           f32CC1sc=-2^31;
      |           warning(['Parameter f32CC1sc of ' gcb ' exceeds the fixed-point range.']);
      |         end
      |         f32CC2sc=round(cc2f*2^(-u16NShiftPI)*2^31);
      |         if f32CC2sc>2^31-1
      |           f32CC2sc=2^31-1;
      |           warning(['Parameter f32CC2sc of ' gcb ' exceeds the fixed-point range.']);
      |         end
      |         if f32CC2sc<-2^31
      |           f32CC2sc=-2^31;
      |           warning(['Parameter f32CC2sc of ' gcb ' exceeds the fixed-point range.']);
      |         end
      |         f32LowerLimit=-2147483648;
      |         f32UpperLimit=2147483647;
      |         c1f=SampleTime*0.5*wmax/3.141592653589793;
      |         u16NShiftI=ceil(log2(abs(c1f)));
      |         if u16NShiftI<0
      |           u16NShiftI=0;
      |         end
      |         if u16NShiftI>31
      |           u16NShiftI=31;
      |           warning(['Parameter u16NShiftI of ' gcb ' exceeds the fixed-point range.']);
      |         end
      |         f32C1=round(c1f*2^(-u16NShiftI)*2^31);
      |         if f32C1>2^31-1
      |           f32C1=2^31-1;
      |           warning(['Parameter f32C1 of ' gcb ' exceeds the fixed-point range.']);
      |         end
      |         if f32C1<-2^31
      |           f32C1=-2^31;
      |           warning(['Parameter f32C1 of ' gcb ' exceeds the fixed-point range.']);
      |         end
      |         if isnan(f32CC1sc)
      |           if ~strcmp(f32CC1sc_bkup,'0')
      |             set_param(gcb,'f32CC1sc','0');
      |           end
      |         else
      |           tmps=num2str(f32CC1sc);
      |           if ~strcmp(f32CC1sc_bkup,tmps)
      |             set_param(gcb,'f32CC1sc',tmps);
      |           end
      |         end
      |         if isnan(f32CC2sc)
      |           if ~strcmp(f32CC2sc_bkup,'0')
      |             set_param(gcb,'f32CC2sc','0');
      |           end
      |         else
      |           tmps=num2str(f32CC2sc);
      |           if ~strcmp(f32CC2sc_bkup,tmps)
      |             set_param(gcb,'f32CC2sc',tmps);
      |           end
      |         end
      |         if isnan(f32UpperLimit)
      |           if ~strcmp(f32UpperLimit_bkup,'0')
      |             set_param(gcb,'f32UpperLimit','0');
      |           end
      |         else
      |           tmps=num2str(f32UpperLimit);
      |           if ~strcmp(f32UpperLimit_bkup,tmps)
      |             set_param(gcb,'f32UpperLimit',tmps);
      |           end
      |         end
      |         if isnan(f32LowerLimit)
      |           if ~strcmp(f32LowerLimit_bkup,'0')
      |             set_param(gcb,'f32LowerLimit','0');
      |           end
      |         else
      |           tmps=num2str(f32LowerLimit);
      |           if ~strcmp(f32LowerLimit_bkup,tmps)
      |             set_param(gcb,'f32LowerLimit',tmps);
      |           end
      |         end
      |         if isnan(u16NShiftPI)
      |           if ~strcmp(u16NShiftPI_bkup,'0')
      |             set_param(gcb,'u16NShiftPI','0');
      |           end
      |         else
      |           tmps=num2str(u16NShiftPI);
      |           if ~strcmp(u16NShiftPI_bkup,tmps)
      |             set_param(gcb,'u16NShiftPI',tmps);
      |           end
      |         end
      |         if isnan(f32C1)
      |           if ~strcmp(f32C1_bkup,'0')
      |             set_param(gcb,'f32C1','0');
      |           end
      |         else
      |           tmps=num2str(f32C1);
      |           if ~strcmp(f32C1_bkup,tmps)
      |             set_param(gcb,'f32C1',tmps);
      |           end
      |         end
      |         if isnan(u16NShiftI)
      |           if ~strcmp(u16NShiftI_bkup,'0')
      |             set_param(gcb,'u16NShiftI','0');
      |           end
      |         else
      |           tmps=num2str(u16NShiftI);
      |           if ~strcmp(u16NShiftI_bkup,tmps)
      |             set_param(gcb,'u16NShiftI',tmps);
      |           end
      |         end
      |       end
      |     end
      |   catch
      |    warning(['Sample time cannot be calculated for the block ' gcb])
      |   end
      | end
      mask DialogControl timeHint Prompt: Note: Implementation parameters cannot be calculated yet because the block's inherited sample time is unknown. Simulink will update the sample time when you run the simulation.
      mask Display:
      | color('black');
      | pos = get_param(gcb, 'Position');
      | width = pos(3) - pos(1);
      | height = pos(4) - pos(2);
      | tX=width/2;
      | tY=height - 25;
      | color('black');
      | text(tX,tY, 'AMCLIB_TrackObsrv_F32', 'horizontalAlignment', 'center');
      | if showStates == 2
      |   color('red');
      |   text(tX,tY - 20, ['debugging mode' char(13) char(10) '(limited performance)'], 'horizontalAlignment', 'center');
      | end
  AMCLIB_Windmilling_F32 : Subsystem  StartFcn=|  TreatAsAtomicUnit=on  mask(AMCLIB_Windmilling_F32){showStates=Hide (faster execution), SampleTime=-1, if0=350, iksi=1, mechspeed=3000, polepairs=1, ADCMaxError=0.002, uscale=12, autoCalcEn=on, f32ADCMaxError=0, f32CC1sc=0, f32CC2sc=0, f32UpperLimit=0, f32LowerLimit=0, u16NShiftPI=0, f32C1=0, u16NShiftI=0, SampleTime_1=NaN}
      | ts=get_param(gcb,'CompiledSampleTime');
      | if iscell(ts)
      |   ts=ts{1};
      |   if iscell(ts)
      |     ts=ts{1};
      |   end
      | end
      | ts=ts(1);
      | set_param(gcb,'SampleTime_1',num2str(ts));
      | p=Simulink.Mask.get(gcb);
      | hintText=p.getDialogControl('timeHint');
      | SampleTime=Simulink.data.evalinGlobal(bdroot,get_param(gcb,'SampleTime'));
      | p=Simulink.Mask.get(gcb);
      | autoCalcEn=get_param(gcb,'autoCalcEn');
      | if strcmp(autoCalcEn,'on')
      |   if SampleTime==-1
      |     hintText.Prompt='Caution: Implementation parameters depend on inherited sample time. Make sure that the sample time of the block''s inputs corresponds to the sampling period in the target application.';
      |   else
      |     hintText.Prompt='Caution: Implementation parameters depend on the sample time. Make sure that the simulation time step corresponds to the sampling period in the target application.';
      |   end
      |   SampleTime=ts;
      |   f32ADCMaxError_bkup=get_param(gcb,'f32ADCMaxError');
      |   f32CC1sc_bkup=get_param(gcb,'f32CC1sc');
      |   f32CC2sc_bkup=get_param(gcb,'f32CC2sc');
      |   f32UpperLimit_bkup=get_param(gcb,'f32UpperLimit');
      |   f32LowerLimit_bkup=get_param(gcb,'f32LowerLimit');
      |   u16NShiftPI_bkup=get_param(gcb,'u16NShiftPI');
      |   f32C1_bkup=get_param(gcb,'f32C1');
      |   u16NShiftI_bkup=get_param(gcb,'u16NShiftI');
      |   if0=Simulink.data.evalinGlobal(bdroot,get_param(gcb,'if0'));
      |   iksi=Simulink.data.evalinGlobal(bdroot,get_param(gcb,'iksi'));
      |   mechspeed=Simulink.data.evalinGlobal(bdroot,get_param(gcb,'mechspeed'));
      |   polepairs=Simulink.data.evalinGlobal(bdroot,get_param(gcb,'polepairs'));
      |   ADCMaxError=Simulink.data.evalinGlobal(bdroot,get_param(gcb,'ADCMaxError'));
      |   uscale=Simulink.data.evalinGlobal(bdroot,get_param(gcb,'uscale'));
      |   if (if0<=0)
      |     warning('Natural frequency f0 must be positive.');
      |   end
      |   if (iksi<=0)
      |     warning('Feedback loop attenuation must be positive.');
      |   end
      |   if (iksi>1)
      |     warning('Feedback loop attenuation must not exceed 1.');
      |   end
      |   if (mechspeed<=0)
      |     warning('Max. speed must be positive.');
      |   end
      |   if (polepairs<1)
      |     warning('Number of pole pairs must be a natural number (1, 2, 3, ...).');
      |   end
      |   if (round(polepairs)~=polepairs)
      |     warning('Number of pole pairs must be a natural number (1, 2, 3, ...).');
      |   end
      |   if (ADCMaxError<=0)
      |     warning('f32ADCMaxError must be positive.');
      |   end
      |   adcsc=ADCMaxError/uscale;
      |   f32ADCMaxError=round(adcsc*2^31);
      |   if f32ADCMaxError>2^31-1
      |     f32ADCMaxError=2^31-1;
      |     warning(['Parameter f32ADCMaxError of ' gcb ' exceeds the fixed-point range.']);
      |   end
      |   if f32ADCMaxError<-2^31
      |     f32ADCMaxError=-2^31;
      |     warning(['Parameter f32ADCMaxError of ' gcb ' exceeds the fixed-point range.']);
      |   end
      |   pgain=12.56637061435917*iksi*if0;
      |   igain=39.47841760435743*if0*if0;
      |   cc1=pgain+igain*SampleTime*0.5;
      |   cc2=-pgain+igain*SampleTime*0.5;
      |   wmax=polepairs*mechspeed*0.1047197551196598;
      |   cc1f=cc1*3.141592653589793/wmax;
      |   cc2f=cc2*3.141592653589793/wmax;
      |   u16NShiftPI=ceil(log2(abs(cc1f)));
      |   tmpsh=ceil(log2(abs(cc2f)));
      |   if u16NShiftPI<tmpsh
      |     u16NShiftPI=tmpsh;
      |   end
      |   if u16NShiftPI<0
      |     u16NShiftPI=0;
      |   end
      |   if u16NShiftPI>31
      |     u16NShiftPI=31;
      |     warning(['Parameter u16NShiftPI of ' gcb ' exceeds the fixed-point range.']);
      |   end
      |   f32CC1sc=round(cc1f*2^(-u16NShiftPI)*2^31);
      |   if f32CC1sc>2^31-1
      |     f32CC1sc=2^31-1;
      |     warning(['Parameter f32CC1sc of ' gcb ' exceeds the fixed-point range.']);
      |   end
      |   if f32CC1sc<-2^31
      |     f32CC1sc=-2^31;
      |     warning(['Parameter f32CC1sc of ' gcb ' exceeds the fixed-point range.']);
      |   end
      |   f32CC2sc=round(cc2f*2^(-u16NShiftPI)*2^31);
      |   if f32CC2sc>2^31-1
      |     f32CC2sc=2^31-1;
      |     warning(['Parameter f32CC2sc of ' gcb ' exceeds the fixed-point range.']);
      |   end
      |   if f32CC2sc<-2^31
      |     f32CC2sc=-2^31;
      |     warning(['Parameter f32CC2sc of ' gcb ' exceeds the fixed-point range.']);
      |   end
      |   f32LowerLimit=-2147483648;
      |   f32UpperLimit=2147483647;
      |   c1f=SampleTime*0.5*wmax/3.141592653589793;
      |   u16NShiftI=ceil(log2(abs(c1f)));
      |   if u16NShiftI<0
      |     u16NShiftI=0;
      |   end
      |   if u16NShiftI>31
      |     u16NShiftI=31;
      |     warning(['Parameter u16NShiftI of ' gcb ' exceeds the fixed-point range.']);
      |   end
      |   f32C1=round(c1f*2^(-u16NShiftI)*2^31);
      |   if f32C1>2^31-1
      |     f32C1=2^31-1;
      |     warning(['Parameter f32C1 of ' gcb ' exceeds the fixed-point range.']);
      |   end
      |   if f32C1<-2^31
      |     f32C1=-2^31;
      |     warning(['Parameter f32C1 of ' gcb ' exceeds the fixed-point range.']);
      |   end
      |   if isnan(f32ADCMaxError)
      |     if ~strcmp(f32ADCMaxError_bkup,'0')
      |       set_param(gcb,'f32ADCMaxError','0');
      |     end
      |   else
      |     tmps=num2str(f32ADCMaxError);
      |     if ~strcmp(f32ADCMaxError_bkup,tmps)
      |       set_param(gcb,'f32ADCMaxError',tmps);
      |     end
      |   end
      |   if isnan(f32CC1sc)
      |     if ~strcmp(f32CC1sc_bkup,'0')
      |       set_param(gcb,'f32CC1sc','0');
      |     end
      |   else
      |     tmps=num2str(f32CC1sc);
      |     if ~strcmp(f32CC1sc_bkup,tmps)
      |       set_param(gcb,'f32CC1sc',tmps);
      |     end
      |   end
      |   if isnan(f32CC2sc)
      |     if ~strcmp(f32CC2sc_bkup,'0')
      |       set_param(gcb,'f32CC2sc','0');
      |     end
      |   else
      |     tmps=num2str(f32CC2sc);
      |     if ~strcmp(f32CC2sc_bkup,tmps)
      |       set_param(gcb,'f32CC2sc',tmps);
      |     end
      |   end
      |   if isnan(f32UpperLimit)
      |     if ~strcmp(f32UpperLimit_bkup,'0')
      |       set_param(gcb,'f32UpperLimit','0');
      |     end
      |   else
      |     tmps=num2str(f32UpperLimit);
      |     if ~strcmp(f32UpperLimit_bkup,tmps)
      |       set_param(gcb,'f32UpperLimit',tmps);
      |     end
      |   end
      |   if isnan(f32LowerLimit)
      |     if ~strcmp(f32LowerLimit_bkup,'0')
      |       set_param(gcb,'f32LowerLimit','0');
      |     end
      |   else
      |     tmps=num2str(f32LowerLimit);
      |     if ~strcmp(f32LowerLimit_bkup,tmps)
      |       set_param(gcb,'f32LowerLimit',tmps);
      |     end
      |   end
      |   if isnan(u16NShiftPI)
      |     if ~strcmp(u16NShiftPI_bkup,'0')
      |       set_param(gcb,'u16NShiftPI','0');
      |     end
      |   else
      |     tmps=num2str(u16NShiftPI);
      |     if ~strcmp(u16NShiftPI_bkup,tmps)
      |       set_param(gcb,'u16NShiftPI',tmps);
      |     end
      |   end
      |   if isnan(f32C1)
      |     if ~strcmp(f32C1_bkup,'0')
      |       set_param(gcb,'f32C1','0');
      |     end
      |   else
      |     tmps=num2str(f32C1);
      |     if ~strcmp(f32C1_bkup,tmps)
      |       set_param(gcb,'f32C1',tmps);
      |     end
      |   end
      |   if isnan(u16NShiftI)
      |     if ~strcmp(u16NShiftI_bkup,'0')
      |       set_param(gcb,'u16NShiftI','0');
      |     end
      |   else
      |     tmps=num2str(u16NShiftI);
      |     if ~strcmp(u16NShiftI_bkup,tmps)
      |       set_param(gcb,'u16NShiftI',tmps);
      |     end
      |   end
      | end
      mask prompts: showStates "Show internal states:"; SampleTime "Sample time (-1 for inherited):"; if0 "Feedback loop natural frequency f0 [Hz]:"; iksi "Feedback loop attenuation ξ:"; mechspeed "Maximum mechanical speed of the motor [RPM]:"; polepairs "Number of pole pairs of the motor:"; ADCMaxError "Maximum differential offset error between any two
phases of the 3-phase voltage-sensing A/D converters [V]:"; uscale "U_max (maximum DC bus voltage) [V]:"; autoCalcEn "Calculate implementation parameters from physical parameters"; f32ADCMaxError "f32ADCMaxError (Max. ADC differential offset error):"; f32CC1sc "f32CC1sc (GFLIB_ControllerPIrAW - CC1 coefficient):"; f32CC2sc "f32CC2sc (GFLIB_ControllerPIrAW - CC2 coefficient):"; f32UpperLimit "f32UpperLimit (GFLIB_ControllerPIrAW - upper Limit of the controller):"; f32LowerLimit "f32LowerLimit (GFLIB_ControllerPIrAW - lower Limit of the controller):"; u16NShiftPI "u16NShiftPI (GFLIB_ControllerPIrAW - scaling
bitwise shift applied to the controller coefficients):"; f32C1 "f32C1 (GFLIB_IntegratorTR - integrator coefficient):"; u16NShiftI "u16NShiftI (GFLIB_IntegratorTR - scaling
bitwise shift applied to the integrator coefficient):"; SampleTime_1 "Discrete sample time:"
      mask help: PMSM Windmilling in 32-bit fixed-point fractional implementation. This function detects spontaneous rotation of an unpowered 3-phase PMSM by measuring the generated back electromotive force. Output u32Lock represents the return value of the C function (0 = undecided, 1 = spinning, 2 = stopped). Transition from 0 to 1 on the u32Lock output can be taken as a reset signal for the following AMCLIB_TrackObsrv_F32 block to synchronize the sensorless FOC loop with a freewheeling motor. Refer to the AMMCLIB User's Guide for further details.
      mask init:
      | ddName = get_param(bdroot,'DataDictionary');
      | if length(ddName)==0
      |   set_param(bdroot,'DataDictionary','ammclib_types.sldd');
      | else
      |   dd = Simulink.data.dictionary.open(ddName);
      |   data = getSection(dd,'Design Data');
      |   if ~exist(data,'SWLIBS_2Syst_F16')
      |     addDataSource(dd,'ammclib_types.sldd');
      |     saveChanges(dd);
      |   end
      | end
      | 
      | if showStates == 1
      |   % hidden state variables
      |   if strcmp(get_param([gcb '/f32ADCMaxError'], 'BlockType'), 'Inport')
      |     posblk = get_param(gcb, 'Position');
      | 
      |     pos = get_param([gcb, '/f32ADCMaxError'], 'Position');
      |     orient = get_param([gcb, '/f32ADCMaxError'], 'Orientation');
      |     delete_block([gcb, '/f32ADCMaxError']);
      |     add_block('built-in/Ground', [gcb, '/f32ADCMaxError'], 'Position', pos, 'Orientation', orient);
      | 
      |     pos = get_param([gcb, '/f32CC1sc'], 'Position');
      |     orient = get_param([gcb, '/f32CC1sc'], 'Orientation');
      |     delete_block([gcb, '/f32CC1sc']);
      |     add_block('built-in/Ground', [gcb, '/f32CC1sc'], 'Position', pos, 'Orientation', orient);
      | 
      |     pos = get_param([gcb, '/f32CC2sc'], 'Position');
      |     orient = get_param([gcb, '/f32CC2sc'], 'Orientation');
      |     delete_block([gcb, '/f32CC2sc']);
      |     add_block('built-in/Ground', [gcb, '/f32CC2sc'], 'Position', pos, 'Orientation', orient);
      | 
      |     pos = get_param([gcb, '/f32UpperLimit'], 'Position');
      |     orient = get_param([gcb, '/f32UpperLimit'], 'Orientation');
      |     delete_block([gcb, '/f32UpperLimit']);
      |     add_block('built-in/Ground', [gcb, '/f32UpperLimit'], 'Position', pos, 'Orientation', orient);
      | 
      |     pos = get_param([gcb, '/f32LowerLimit'], 'Position');
      |     orient = get_param([gcb, '/f32LowerLimit'], 'Orientation');
      |     delete_block([gcb, '/f32LowerLimit']);
      |     add_block('built-in/Ground', [gcb, '/f32LowerLimit'], 'Position', pos, 'Orientation', orient);
      | 
      |     pos = get_param([gcb, '/u16NShiftPI'], 'Position');
      |     orient = get_param([gcb, '/u16NShiftPI'], 'Orientation');
      |     delete_block([gcb, '/u16NShiftPI']);
      |     add_block('built-in/Ground', [gcb, '/u16NShiftPI'], 'Position', pos, 'Orientation', orient);
      | 
      |     pos = get_param([gcb, '/f32C1'], 'Position');
      |     orient = get_param([gcb, '/f32C1'], 'Orientation');
      |     delete_block([gcb, '/f32C1']);
      |     add_block('built-in/Ground', [gcb, '/f32C1'], 'Position', pos, 'Orientation', orient);
      | 
      |     pos = get_param([gcb, '/u16NShiftI'], 'Position');
      |     orient = get_param([gcb, '/u16NShiftI'], 'Orientation');
      |     delete_block([gcb, '/u16NShiftI']);
      |     add_block('built-in/Ground', [gcb, '/u16NShiftI'], 'Position', pos, 'Orientation', orient);
      | 
      |     pos = get_param([gcb, '/f32AccPI'], 'Position');
      |     orient = get_param([gcb, '/f32AccPI'], 'Orientation');
      |     delete_block([gcb, '/f32AccPI']);
      |     add_block('built-in/Ground', [gcb, '/f32AccPI'], 'Position', pos, 'Orientation', orient);
      | 
      |     pos = get_param([gcb, '/f32InErrK1'], 'Position');
      |     orient = get_param([gcb, '/f32InErrK1'], 'Orientation');
      |     delete_block([gcb, '/f32InErrK1']);
      |     add_block('built-in/Ground', [gcb, '/f32InErrK1'], 'Position', pos, 'Orientation', orient);
      | 
      |     pos = get_param([gcb, '/f32State'], 'Position');
      |     orient = get_param([gcb, '/f32State'], 'Orientation');
      |     delete_block([gcb, '/f32State']);
      |     add_block('built-in/Ground', [gcb, '/f32State'], 'Position', pos, 'Orientation', orient);
      | 
      |     pos = get_param([gcb, '/f32InK1'], 'Position');
      |     orient = get_param([gcb, '/f32InK1'], 'Orientation');
      |     delete_block([gcb, '/f32InK1']);
      |     add_block('built-in/Ground', [gcb, '/f32InK1'], 'Position', pos, 'Orientation', orient);
      | 
      | 
      |     pmask=Simulink.Mask.get(gcb);
      |     pctrl=pmask.getParameter('SampleTime');
      |     pctrl.set('TypeOptions',{'pUabcIn/SampleTime'});
      | 
      |     pos = get_param([gcb '/f32AccPI_Out'], 'Position');
      |     orient = get_param([gcb '/f32AccPI_Out'], 'Orientation');
      |     delete_block([gcb '/f32AccPI_Out']);
      |     add_block('built-in/Terminator', [gcb '/f32AccPI_Out'], 'Position', pos, 'Orientation', orient);
      | 
      |     pos = get_param([gcb '/f32InErrK1_Out'], 'Position');
      |     orient = get_param([gcb '/f32InErrK1_Out'], 'Orientation');
      |     delete_block([gcb '/f32InErrK1_Out']);
      |     add_block('built-in/Terminator', [gcb '/f32InErrK1_Out'], 'Position', pos, 'Orientation', orient);
      | 
      |     pos = get_param([gcb '/f32State_Out'], 'Position');
      |     orient = get_param([gcb '/f32State_Out'], 'Orientation');
      |     delete_block([gcb '/f32State_Out']);
      |     add_block('built-in/Terminator', [gcb '/f32State_Out'], 'Position', pos, 'Orientation', orient);
      | 
      |     pos = get_param([gcb '/f32InK1_Out'], 'Position');
      |     orient = get_param([gcb '/f32InK1_Out'], 'Orientation');
      |     delete_block([gcb '/f32InK1_Out']);
      |     add_block('built-in/Terminator', [gcb '/f32InK1_Out'], 'Position', pos, 'Orientation', orient);
      | 
      |     set_param([gcb '/pUabcIn'], 'Port', '1');
      | 
      |     tmpOutCnt=0;
      |     tmpOutCnt=tmpOutCnt+1;
      |     set_param([gcb '/u32Lock'], 'Port', num2str(tmpOutCnt));
      |     tmpOutCnt=tmpOutCnt+1;
      |     set_param([gcb '/pPosEst'], 'Port', num2str(tmpOutCnt));
      |     tmpOutCnt=tmpOutCnt+1;
      |     set_param([gcb '/pVelocityEst'], 'Port', num2str(tmpOutCnt));
      | 
      |     autoCalcEn=get_param(gcb,'autoCalcEn');
      |     if strcmp(autoCalcEn,'on')
      |       set_param(gcb,'MaskEnables',{'on','on','on','on','on','on','on','on','on','on','on','on','on','on','on','on','on','off'});
      |     else
      |       set_param(gcb,'MaskEnables',{'on','on','off','off','off','off','off','off','on','on','on','on','on','on','on','on','on','off'});
      |     end
      | 
      |     if (posblk(4) - posblk(2)) > 100
      |       height = 100;
      |       set_param(gcb,'Position',[posblk(1), posblk(2), posblk(3), posblk(2)+height])
      |     end
      |   end
      | else
      |   % shown state variables
      |   if strcmp(get_param([gcb '/f32ADCMaxError'], 'BlockType'), 'Ground')
      |     posblk = get_param(gcb, 'Position');
      | 
      |     pos = get_param([gcb, '/f32ADCMaxError'], 'Position');
      |     orient = get_param([gcb, '/f32ADCMaxError'], 'Orientation');
      |     delete_block([gcb, '/f32ADCMaxError']);
      |     add_block('built-in/Inport', [gcb, '/f32ADCMaxError'], 'Position', pos, 'Orientation', orient, 'OutDataTypeStr', 'int32');
      | 
      |     pos = get_param([gcb, '/f32CC1sc'], 'Position');
      |     orient = get_param([gcb, '/f32CC1sc'], 'Orientation');
      |     delete_block([gcb, '/f32CC1sc']);
      |     add_block('built-in/Inport', [gcb, '/f32CC1sc'], 'Position', pos, 'Orientation', orient, 'OutDataTypeStr', 'int32');
      | 
      |     pos = get_param([gcb, '/f32CC2sc'], 'Position');
      |     orient = get_param([gcb, '/f32CC2sc'], 'Orientation');
      |     delete_block([gcb, '/f32CC2sc']);
      |     add_block('built-in/Inport', [gcb, '/f32CC2sc'], 'Position', pos, 'Orientation', orient, 'OutDataTypeStr', 'int32');
      | 
      |     pos = get_param([gcb, '/f32UpperLimit'], 'Position');
      |     orient = get_param([gcb, '/f32UpperLimit'], 'Orientation');
      |     delete_block([gcb, '/f32UpperLimit']);
      |     add_block('built-in/Inport', [gcb, '/f32UpperLimit'], 'Position', pos, 'Orientation', orient, 'OutDataTypeStr', 'int32');
      | 
      |     pos = get_param([gcb, '/f32LowerLimit'], 'Position');
      |     orient = get_param([gcb, '/f32LowerLimit'], 'Orientation');
      |     delete_block([gcb, '/f32LowerLimit']);
      |     add_block('built-in/Inport', [gcb, '/f32LowerLimit'], 'Position', pos, 'Orientation', orient, 'OutDataTypeStr', 'int32');
      | 
      |     pos = get_param([gcb, '/u16NShiftPI'], 'Position');
      |     orient = get_param([gcb, '/u16NShiftPI'], 'Orientation');
      |     delete_block([gcb, '/u16NShiftPI']);
      |     add_block('built-in/Inport', [gcb, '/u16NShiftPI'], 'Position', pos, 'Orientation', orient, 'OutDataTypeStr', 'uint16');
      | 
      |     pos = get_param([gcb, '/f32C1'], 'Position');
      |     orient = get_param([gcb, '/f32C1'], 'Orientation');
      |     delete_block([gcb, '/f32C1']);
      |     add_block('built-in/Inport', [gcb, '/f32C1'], 'Position', pos, 'Orientation', orient, 'OutDataTypeStr', 'int32');
      | 
      |     pos = get_param([gcb, '/u16NShiftI'], 'Position');
      |     orient = get_param([gcb, '/u16NShiftI'], 'Orientation');
      |     delete_block([gcb, '/u16NShiftI']);
      |     add_block('built-in/Inport', [gcb, '/u16NShiftI'], 'Position', pos, 'Orientation', orient, 'OutDataTypeStr', 'uint16');
      | 
      |     pos = get_param([gcb, '/f32AccPI'], 'Position');
      |     orient = get_param([gcb, '/f32AccPI'], 'Orientation');
      |     delete_block([gcb, '/f32AccPI']);
      |     add_block('built-in/Inport', [gcb, '/f32AccPI'], 'Position', pos, 'Orientation', orient, 'OutDataTypeStr', 'int32');
      | 
      |     pos = get_param([gcb, '/f32InErrK1'], 'Position');
      |     orient = get_param([gcb, '/f32InErrK1'], 'Orientation');
      |     delete_block([gcb, '/f32InErrK1']);
      |     add_block('built-in/Inport', [gcb, '/f32InErrK1'], 'Position', pos, 'Orientation', orient, 'OutDataTypeStr', 'int32');
      | 
      |     pos = get_param([gcb, '/f32State'], 'Position');
      |     orient = get_param([gcb, '/f32State'], 'Orientation');
      |     delete_block([gcb, '/f32State']);
      |     add_block('built-in/Inport', [gcb, '/f32State'], 'Position', pos, 'Orientation', orient, 'OutDataTypeStr', 'int32');
      | 
      |     pos = get_param([gcb, '/f32InK1'], 'Position');
      |     orient = get_param([gcb, '/f32InK1'], 'Orientation');
      |     delete_block([gcb, '/f32InK1']);
      |     add_block('built-in/Inport', [gcb, '/f32InK1'], 'Position', pos, 'Orientation', orient, 'OutDataTypeStr', 'int32');
      | 
      | 
      | 
      |     pos = get_param([gcb '/f32AccPI_Out'], 'Position');
      |     orient = get_param([gcb '/f32AccPI_Out'], 'Orientation');
      |     delete_block([gcb '/f32AccPI_Out']);
      |     add_block('built-in/Outport', [gcb '/f32AccPI_Out'], 'Position', pos, 'Orientation', orient);
      | 
      |     pos = get_param([gcb '/f32InErrK1_Out'], 'Position');
      |     orient = get_param([gcb '/f32InErrK1_Out'], 'Orientation');
      |     delete_block([gcb '/f32InErrK1_Out']);
      |     add_block('built-in/Outport', [gcb '/f32InErrK1_Out'], 'Position', pos, 'Orientation', orient);
      | 
      |     pos = get_param([gcb '/f32State_Out'], 'Position');
      |     orient = get_param([gcb '/f32State_Out'], 'Orientation');
      |     delete_block([gcb '/f32State_Out']);
      |     add_block('built-in/Outport', [gcb '/f32State_Out'], 'Position', pos, 'Orientation', orient);
      | 
      |     pos = get_param([gcb '/f32InK1_Out'], 'Position');
      |     orient = get_param([gcb '/f32InK1_Out'], 'Orientation');
      |     delete_block([gcb '/f32InK1_Out']);
      |     add_block('built-in/Outport', [gcb '/f32InK1_Out'], 'Position', pos, 'Orientation', orient);
      | 
      | 
      |     pmask=Simulink.Mask.get(gcb);
      |     pctrl=pmask.getParameter('SampleTime');
      |     pctrl.set('TypeOptions',{'pUabcIn/SampleTime','f32ADCMaxError/SampleTime','f32CC1sc/SampleTime','f32CC2sc/SampleTime','f32UpperLimit/SampleTime','f32LowerLimit/SampleTime','u16NShiftPI/SampleTime','f32C1/SampleTime','u16NShiftI/SampleTime','f32AccPI/SampleTime','f32InErrK1/SampleTime','f32State/SampleTime','f32InK1/SampleTime'});
      | 
      |     set_param([gcb '/pUabcIn'], 'Port', '1');
      |     set_param([gcb '/f32ADCMaxError'], 'Port', '2');
      |     set_param([gcb '/f32CC1sc'], 'Port', '3');
      |     set_param([gcb '/f32CC2sc'], 'Port', '4');
      |     set_param([gcb '/f32UpperLimit'], 'Port', '5');
      |     set_param([gcb '/f32LowerLimit'], 'Port', '6');
      |     set_param([gcb '/u16NShiftPI'], 'Port', '7');
      |     set_param([gcb '/f32C1'], 'Port', '8');
      |     set_param([gcb '/u16NShiftI'], 'Port', '9');
      |     set_param([gcb '/f32AccPI'], 'Port', '10');
      |     set_param([gcb '/f32InErrK1'], 'Port', '11');
      |     set_param([gcb '/f32State'], 'Port', '12');
      |     set_param([gcb '/f32InK1'], 'Port', '13');
      | 
      |     tmpOutCnt=0;
      |     tmpOutCnt=tmpOutCnt+1;
      |     set_param([gcb '/u32Lock'], 'Port', num2str(tmpOutCnt));
      |     tmpOutCnt=tmpOutCnt+1;
      |     set_param([gcb '/pPosEst'], 'Port', num2str(tmpOutCnt));
      |     tmpOutCnt=tmpOutCnt+1;
      |     set_param([gcb '/pVelocityEst'], 'Port', num2str(tmpOutCnt));
      |     tmpOutCnt=tmpOutCnt+1;
      |     set_param([gcb '/f32AccPI_Out'], 'Port', num2str(tmpOutCnt));
      |     tmpOutCnt=tmpOutCnt+1;
      |     set_param([gcb '/f32InErrK1_Out'], 'Port', num2str(tmpOutCnt));
      |     tmpOutCnt=tmpOutCnt+1;
      |     set_param([gcb '/f32State_Out'], 'Port', num2str(tmpOutCnt));
      |     tmpOutCnt=tmpOutCnt+1;
      |     set_param([gcb '/f32InK1_Out'], 'Port', num2str(tmpOutCnt));
      | 
      |     set_param(gcb,'MaskEnables',{'on','on','off','off','off','off','off','off','off','off','off','off','off','off','off','off','off','off'});
      | 
      |     if (posblk(4) - posblk(2)) < 350
      |       height = 350;
      |       set_param(gcb,'Position',[posblk(1), posblk(2), posblk(3), posblk(2)+height])
      |     end
      |   end
      | end
      settings: RTWSystemCode=Inline
      mask Help: web([fileparts(which('ammclib_bam_S32K3xx.slx')) '/../doc/S32K3XXMCLUG.pdf'], '-browser')
      mask TypeOptions showStates: Hide (faster execution) | Show (allows debugging; connect feedback loops manually)
      mask Callback showStates:
      | maskStr=get_param(gcb,'showStates');
      | if strcmp(maskStr,'Hide (faster execution)')
      |   if strcmp(get_param([gcb '/f32ADCMaxError'], 'BlockType'), 'Inport')
      |     autoCalcEn=get_param(gcb,'autoCalcEn');
      |     if strcmp(autoCalcEn,'on')
      |       set_param(gcb,'MaskEnables',{'on','on','on','on','on','on','on','on','on','on','on','on','on','on','on','on','on','off'});
      |     else
      |       set_param(gcb,'MaskEnables',{'on','on','off','off','off','off','off','off','on','on','on','on','on','on','on','on','on','off'});
      |     end
      |   end
      | else
      |   if strcmp(get_param([gcb '/f32ADCMaxError'], 'BlockType'), 'Ground')
      |     set_param(gcb,'MaskEnables',{'on','on','off','off','off','off','off','off','off','off','off','off','off','off','off','off','off','off'});
      |   end
      | end
      mask TypeOptions SampleTime: pUabcIn/SampleTime
      mask Callback SampleTime:
      | p=Simulink.Mask.get(gcb);
      | hintText=p.getDialogControl('timeHint');
      | SampleTime=Simulink.data.evalinGlobal(bdroot,get_param(gcb,'SampleTime'));
      | SampleTime_1=str2double(get_param(gcb,'SampleTime_1'));
      | if (((SampleTime==-1) && (~contains(hintText.Prompt,'inherited'))) || ...
      |     ((SampleTime~=-1) && contains(hintText.Prompt,'inherited')) || ...
      |     ((SampleTime~=-1) && (SampleTime_1~=SampleTime)) || ...
      |     ((SampleTime_1~=-1) && contains(hintText.Prompt,'yet')))
      |   if ((SampleTime==-1) && (~contains(hintText.Prompt,'inherited')))
      |     set_param(gcb,'SampleTime_1',num2str(NaN));
      |     SampleTime_1=NaN;
      |   end
      |   if (SampleTime~=-1)
      |     set_param(gcb,'SampleTime_1',num2str(SampleTime));
      |     SampleTime_1=SampleTime;
      |   end
      |   autoCalcEn=get_param(gcb,'autoCalcEn');
      |   if strcmp(autoCalcEn,'on')
      |     p=Simulink.Mask.get(gcb);
      |     hintText=p.getDialogControl('timeHint');
      |     if SampleTime==-1
      |       SampleTime=SampleTime_1;
      |       if isnan(SampleTime)
      |         hintText.Prompt='Note: Implementation parameters cannot be calculated yet because the block''s inherited sample time is unknown. Simulink will update the sample time when you run the simulation.';
      |       else
      |         hintText.Prompt='Caution: Implementation parameters depend on inherited sample time. Make sure that the sample time of the block''s inputs corresponds to the sampling period in the target application.';
      |       end
      |     else
      |       hintText.Prompt='Caution: Implementation parameters depend on the sample time. Make sure that the simulation time step corresponds to the sampling period in the target application.';
      |     end
      |     f32ADCMaxError_bkup=get_param(gcb,'f32ADCMaxError');
      |     f32CC1sc_bkup=get_param(gcb,'f32CC1sc');
      |     f32CC2sc_bkup=get_param(gcb,'f32CC2sc');
      |     f32UpperLimit_bkup=get_param(gcb,'f32UpperLimit');
      |     f32LowerLimit_bkup=get_param(gcb,'f32LowerLimit');
      |     u16NShiftPI_bkup=get_param(gcb,'u16NShiftPI');
      |     f32C1_bkup=get_param(gcb,'f32C1');
      |     u16NShiftI_bkup=get_param(gcb,'u16NShiftI');
      |     if0=Simulink.data.evalinGlobal(bdroot,get_param(gcb,'if0'));
      |     iksi=Simulink.data.evalinGlobal(bdroot,get_param(gcb,'iksi'));
      |     mechspeed=Simulink.data.evalinGlobal(bdroot,get_param(gcb,'mechspeed'));
      |     polepairs=Simulink.data.evalinGlobal(bdroot,get_param(gcb,'polepairs'));
      |     ADCMaxError=Simulink.data.evalinGlobal(bdroot,get_param(gcb,'ADCMaxError'));
      |     uscale=Simulink.data.evalinGlobal(bdroot,get_param(gcb,'uscale'));
      |     if (if0<=0)
      |       warning('Natural frequency f0 must be positive.');
      |     end
      |     if (iksi<=0)
      |       warning('Feedback loop attenuation must be positive.');
      |     end
      |     if (iksi>1)
      |       warning('Feedback loop attenuation must not exceed 1.');
      |     end
      |     if (mechspeed<=0)
      |       warning('Max. speed must be positive.');
      |     end
      |     if (polepairs<1)
      |       warning('Number of pole pairs must be a natural number (1, 2, 3, ...).');
      |     end
      |     if (round(polepairs)~=polepairs)
      |       warning('Number of pole pairs must be a natural number (1, 2, 3, ...).');
      |     end
      |     if (ADCMaxError<=0)
      |       warning('f32ADCMaxError must be positive.');
      |     end
      |     adcsc=ADCMaxError/uscale;
      |     f32ADCMaxError=round(adcsc*2^31);
      |     if f32ADCMaxError>2^31-1
      |       f32ADCMaxError=2^31-1;
      |       warning(['Parameter f32ADCMaxError of ' gcb ' exceeds the fixed-point range.']);
      |     end
      |     if f32ADCMaxError<-2^31
      |       f32ADCMaxError=-2^31;
      |       warning(['Parameter f32ADCMaxError of ' gcb ' exceeds the fixed-point range.']);
      |     end
      |     pgain=12.56637061435917*iksi*if0;
      |     igain=39.47841760435743*if0*if0;
      |     cc1=pgain+igain*SampleTime*0.5;
      |     cc2=-pgain+igain*SampleTime*0.5;
      |     wmax=polepairs*mechspeed*0.1047197551196598;
      |     cc1f=cc1*3.141592653589793/wmax;
      |     cc2f=cc2*3.141592653589793/wmax;
      |     u16NShiftPI=ceil(log2(abs(cc1f)));
      |     tmpsh=ceil(log2(abs(cc2f)));
      |     if u16NShiftPI<tmpsh
      |       u16NShiftPI=tmpsh;
      |     end
      |     if u16NShiftPI<0
      |       u16NShiftPI=0;
      |     end
      |     if u16NShiftPI>31
      |       u16NShiftPI=31;
      |       warning(['Parameter u16NShiftPI of ' gcb ' exceeds the fixed-point range.']);
      |     end
      |     f32CC1sc=round(cc1f*2^(-u16NShiftPI)*2^31);
      |     if f32CC1sc>2^31-1
      |       f32CC1sc=2^31-1;
      |       warning(['Parameter f32CC1sc of ' gcb ' exceeds the fixed-point range.']);
      |     end
      |     if f32CC1sc<-2^31
      |       f32CC1sc=-2^31;
      |       warning(['Parameter f32CC1sc of ' gcb ' exceeds the fixed-point range.']);
      |     end
      |     f32CC2sc=round(cc2f*2^(-u16NShiftPI)*2^31);
      |     if f32CC2sc>2^31-1
      |       f32CC2sc=2^31-1;
      |       warning(['Parameter f32CC2sc of ' gcb ' exceeds the fixed-point range.']);
      |     end
      |     if f32CC2sc<-2^31
      |       f32CC2sc=-2^31;
      |       warning(['Parameter f32CC2sc of ' gcb ' exceeds the fixed-point range.']);
      |     end
      |     f32LowerLimit=-2147483648;
      |     f32UpperLimit=2147483647;
      |     c1f=SampleTime*0.5*wmax/3.141592653589793;
      |     u16NShiftI=ceil(log2(abs(c1f)));
      |     if u16NShiftI<0
      |       u16NShiftI=0;
      |     end
      |     if u16NShiftI>31
      |       u16NShiftI=31;
      |       warning(['Parameter u16NShiftI of ' gcb ' exceeds the fixed-point range.']);
      |     end
      |     f32C1=round(c1f*2^(-u16NShiftI)*2^31);
      |     if f32C1>2^31-1
      |       f32C1=2^31-1;
      |       warning(['Parameter f32C1 of ' gcb ' exceeds the fixed-point range.']);
      |     end
      |     if f32C1<-2^31
      |       f32C1=-2^31;
      |       warning(['Parameter f32C1 of ' gcb ' exceeds the fixed-point range.']);
      |     end
      |     if isnan(f32ADCMaxError)
      |       if ~strcmp(f32ADCMaxError_bkup,'0')
      |         set_param(gcb,'f32ADCMaxError','0');
      |       end
      |     else
      |       tmps=num2str(f32ADCMaxError);
      |       if ~strcmp(f32ADCMaxError_bkup,tmps)
      |         set_param(gcb,'f32ADCMaxError',tmps);
      |       end
      |     end
      |     if isnan(f32CC1sc)
      |       if ~strcmp(f32CC1sc_bkup,'0')
      |         set_param(gcb,'f32CC1sc','0');
      |       end
      |     else
      |       tmps=num2str(f32CC1sc);
      |       if ~strcmp(f32CC1sc_bkup,tmps)
      |         set_param(gcb,'f32CC1sc',tmps);
      |       end
      |     end
      |     if isnan(f32CC2sc)
      |       if ~strcmp(f32CC2sc_bkup,'0')
      |         set_param(gcb,'f32CC2sc','0');
      |       end
      |     else
      |       tmps=num2str(f32CC2sc);
      |       if ~strcmp(f32CC2sc_bkup,tmps)
      |         set_param(gcb,'f32CC2sc',tmps);
      |       end
      |     end
      |     if isnan(f32UpperLimit)
      |       if ~strcmp(f32UpperLimit_bkup,'0')
      |         set_param(gcb,'f32UpperLimit','0');
      |       end
      |     else
      |       tmps=num2str(f32UpperLimit);
      |       if ~strcmp(f32UpperLimit_bkup,tmps)
      |         set_param(gcb,'f32UpperLimit',tmps);
      |       end
      |     end
      |     if isnan(f32LowerLimit)
      |       if ~strcmp(f32LowerLimit_bkup,'0')
      |         set_param(gcb,'f32LowerLimit','0');
      |       end
      |     else
      |       tmps=num2str(f32LowerLimit);
      |       if ~strcmp(f32LowerLimit_bkup,tmps)
      |         set_param(gcb,'f32LowerLimit',tmps);
      |       end
      |     end
      |     if isnan(u16NShiftPI)
      |       if ~strcmp(u16NShiftPI_bkup,'0')
      |         set_param(gcb,'u16NShiftPI','0');
      |       end
      |     else
      |       tmps=num2str(u16NShiftPI);
      |       if ~strcmp(u16NShiftPI_bkup,tmps)
      |         set_param(gcb,'u16NShiftPI',tmps);
      |       end
      |     end
      |     if isnan(f32C1)
      |       if ~strcmp(f32C1_bkup,'0')
      |         set_param(gcb,'f32C1','0');
      |       end
      |     else
      |       tmps=num2str(f32C1);
      |       if ~strcmp(f32C1_bkup,tmps)
      |         set_param(gcb,'f32C1',tmps);
      |       end
      |     end
      |     if isnan(u16NShiftI)
      |       if ~strcmp(u16NShiftI_bkup,'0')
      |         set_param(gcb,'u16NShiftI','0');
      |       end
      |     else
      |       tmps=num2str(u16NShiftI);
      |       if ~strcmp(u16NShiftI_bkup,tmps)
      |         set_param(gcb,'u16NShiftI',tmps);
      |       end
      |     end
      |   end
      | end
      mask Callback if0:
      | autoCalcEn=get_param(gcb,'autoCalcEn');
      | if strcmp(autoCalcEn,'on')
      |   SampleTime=Simulink.data.evalinGlobal(bdroot,get_param(gcb,'SampleTime'));
      |   if (SampleTime==-1)
      |     SampleTime=str2double(get_param(gcb,'SampleTime_1'));
      |   end
      |   f32ADCMaxError_bkup=get_param(gcb,'f32ADCMaxError');
      |   f32CC1sc_bkup=get_param(gcb,'f32CC1sc');
      |   f32CC2sc_bkup=get_param(gcb,'f32CC2sc');
      |   f32UpperLimit_bkup=get_param(gcb,'f32UpperLimit');
      |   f32LowerLimit_bkup=get_param(gcb,'f32LowerLimit');
      |   u16NShiftPI_bkup=get_param(gcb,'u16NShiftPI');
      |   f32C1_bkup=get_param(gcb,'f32C1');
      |   u16NShiftI_bkup=get_param(gcb,'u16NShiftI');
      |   if0=Simulink.data.evalinGlobal(bdroot,get_param(gcb,'if0'));
      |   iksi=Simulink.data.evalinGlobal(bdroot,get_param(gcb,'iksi'));
      |   mechspeed=Simulink.data.evalinGlobal(bdroot,get_param(gcb,'mechspeed'));
      |   polepairs=Simulink.data.evalinGlobal(bdroot,get_param(gcb,'polepairs'));
      |   ADCMaxError=Simulink.data.evalinGlobal(bdroot,get_param(gcb,'ADCMaxError'));
      |   uscale=Simulink.data.evalinGlobal(bdroot,get_param(gcb,'uscale'));
      |   if (if0<=0)
      |     warning('Natural frequency f0 must be positive.');
      |   end
      |   if (iksi<=0)
      |     warning('Feedback loop attenuation must be positive.');
      |   end
      |   if (iksi>1)
      |     warning('Feedback loop attenuation must not exceed 1.');
      |   end
      |   if (mechspeed<=0)
      |     warning('Max. speed must be positive.');
      |   end
      |   if (polepairs<1)
      |     warning('Number of pole pairs must be a natural number (1, 2, 3, ...).');
      |   end
      |   if (round(polepairs)~=polepairs)
      |     warning('Number of pole pairs must be a natural number (1, 2, 3, ...).');
      |   end
      |   if (ADCMaxError<=0)
      |     warning('f32ADCMaxError must be positive.');
      |   end
      |   adcsc=ADCMaxError/uscale;
      |   f32ADCMaxError=round(adcsc*2^31);
      |   if f32ADCMaxError>2^31-1
      |     f32ADCMaxError=2^31-1;
      |     warning(['Parameter f32ADCMaxError of ' gcb ' exceeds the fixed-point range.']);
      |   end
      |   if f32ADCMaxError<-2^31
      |     f32ADCMaxError=-2^31;
      |     warning(['Parameter f32ADCMaxError of ' gcb ' exceeds the fixed-point range.']);
      |   end
      |   pgain=12.56637061435917*iksi*if0;
      |   igain=39.47841760435743*if0*if0;
      |   cc1=pgain+igain*SampleTime*0.5;
      |   cc2=-pgain+igain*SampleTime*0.5;
      |   wmax=polepairs*mechspeed*0.1047197551196598;
      |   cc1f=cc1*3.141592653589793/wmax;
      |   cc2f=cc2*3.141592653589793/wmax;
      |   u16NShiftPI=ceil(log2(abs(cc1f)));
      |   tmpsh=ceil(log2(abs(cc2f)));
      |   if u16NShiftPI<tmpsh
      |     u16NShiftPI=tmpsh;
      |   end
      |   if u16NShiftPI<0
      |     u16NShiftPI=0;
      |   end
      |   if u16NShiftPI>31
      |     u16NShiftPI=31;
      |     warning(['Parameter u16NShiftPI of ' gcb ' exceeds the fixed-point range.']);
      |   end
      |   f32CC1sc=round(cc1f*2^(-u16NShiftPI)*2^31);
      |   if f32CC1sc>2^31-1
      |     f32CC1sc=2^31-1;
      |     warning(['Parameter f32CC1sc of ' gcb ' exceeds the fixed-point range.']);
      |   end
      |   if f32CC1sc<-2^31
      |     f32CC1sc=-2^31;
      |     warning(['Parameter f32CC1sc of ' gcb ' exceeds the fixed-point range.']);
      |   end
      |   f32CC2sc=round(cc2f*2^(-u16NShiftPI)*2^31);
      |   if f32CC2sc>2^31-1
      |     f32CC2sc=2^31-1;
      |     warning(['Parameter f32CC2sc of ' gcb ' exceeds the fixed-point range.']);
      |   end
      |   if f32CC2sc<-2^31
      |     f32CC2sc=-2^31;
      |     warning(['Parameter f32CC2sc of ' gcb ' exceeds the fixed-point range.']);
      |   end
      |   f32LowerLimit=-2147483648;
      |   f32UpperLimit=2147483647;
      |   c1f=SampleTime*0.5*wmax/3.141592653589793;
      |   u16NShiftI=ceil(log2(abs(c1f)));
      |   if u16NShiftI<0
      |     u16NShiftI=0;
      |   end
      |   if u16NShiftI>31
      |     u16NShiftI=31;
      |     warning(['Parameter u16NShiftI of ' gcb ' exceeds the fixed-point range.']);
      |   end
      |   f32C1=round(c1f*2^(-u16NShiftI)*2^31);
      |   if f32C1>2^31-1
      |     f32C1=2^31-1;
      |     warning(['Parameter f32C1 of ' gcb ' exceeds the fixed-point range.']);
      |   end
      |   if f32C1<-2^31
      |     f32C1=-2^31;
      |     warning(['Parameter f32C1 of ' gcb ' exceeds the fixed-point range.']);
      |   end
      |   if isnan(f32ADCMaxError)
      |     if ~strcmp(f32ADCMaxError_bkup,'0')
      |       set_param(gcb,'f32ADCMaxError','0');
      |     end
      |   else
      |     tmps=num2str(f32ADCMaxError);
      |     if ~strcmp(f32ADCMaxError_bkup,tmps)
      |       set_param(gcb,'f32ADCMaxError',tmps);
      |     end
      |   end
      |   if isnan(f32CC1sc)
      |     if ~strcmp(f32CC1sc_bkup,'0')
      |       set_param(gcb,'f32CC1sc','0');
      |     end
      |   else
      |     tmps=num2str(f32CC1sc);
      |     if ~strcmp(f32CC1sc_bkup,tmps)
      |       set_param(gcb,'f32CC1sc',tmps);
      |     end
      |   end
      |   if isnan(f32CC2sc)
      |     if ~strcmp(f32CC2sc_bkup,'0')
      |       set_param(gcb,'f32CC2sc','0');
      |     end
      |   else
      |     tmps=num2str(f32CC2sc);
      |     if ~strcmp(f32CC2sc_bkup,tmps)
      |       set_param(gcb,'f32CC2sc',tmps);
      |     end
      |   end
      |   if isnan(f32UpperLimit)
      |     if ~strcmp(f32UpperLimit_bkup,'0')
      |       set_param(gcb,'f32UpperLimit','0');
      |     end
      |   else
      |     tmps=num2str(f32UpperLimit);
      |     if ~strcmp(f32UpperLimit_bkup,tmps)
      |       set_param(gcb,'f32UpperLimit',tmps);
      |     end
      |   end
      |   if isnan(f32LowerLimit)
      |     if ~strcmp(f32LowerLimit_bkup,'0')
      |       set_param(gcb,'f32LowerLimit','0');
      |     end
      |   else
      |     tmps=num2str(f32LowerLimit);
      |     if ~strcmp(f32LowerLimit_bkup,tmps)
      |       set_param(gcb,'f32LowerLimit',tmps);
      |     end
      |   end
      |   if isnan(u16NShiftPI)
      |     if ~strcmp(u16NShiftPI_bkup,'0')
      |       set_param(gcb,'u16NShiftPI','0');
      |     end
      |   else
      |     tmps=num2str(u16NShiftPI);
      |     if ~strcmp(u16NShiftPI_bkup,tmps)
      |       set_param(gcb,'u16NShiftPI',tmps);
      |     end
      |   end
      |   if isnan(f32C1)
      |     if ~strcmp(f32C1_bkup,'0')
      |       set_param(gcb,'f32C1','0');
      |     end
      |   else
      |     tmps=num2str(f32C1);
      |     if ~strcmp(f32C1_bkup,tmps)
      |       set_param(gcb,'f32C1',tmps);
      |     end
      |   end
      |   if isnan(u16NShiftI)
      |     if ~strcmp(u16NShiftI_bkup,'0')
      |       set_param(gcb,'u16NShiftI','0');
      |     end
      |   else
      |     tmps=num2str(u16NShiftI);
      |     if ~strcmp(u16NShiftI_bkup,tmps)
      |       set_param(gcb,'u16NShiftI',tmps);
      |     end
      |   end
      | end
      mask Callback iksi:
      | autoCalcEn=get_param(gcb,'autoCalcEn');
      | if strcmp(autoCalcEn,'on')
      |   SampleTime=Simulink.data.evalinGlobal(bdroot,get_param(gcb,'SampleTime'));
      |   if (SampleTime==-1)
      |     SampleTime=str2double(get_param(gcb,'SampleTime_1'));
      |   end
      |   f32ADCMaxError_bkup=get_param(gcb,'f32ADCMaxError');
      |   f32CC1sc_bkup=get_param(gcb,'f32CC1sc');
      |   f32CC2sc_bkup=get_param(gcb,'f32CC2sc');
      |   f32UpperLimit_bkup=get_param(gcb,'f32UpperLimit');
      |   f32LowerLimit_bkup=get_param(gcb,'f32LowerLimit');
      |   u16NShiftPI_bkup=get_param(gcb,'u16NShiftPI');
      |   f32C1_bkup=get_param(gcb,'f32C1');
      |   u16NShiftI_bkup=get_param(gcb,'u16NShiftI');
      |   if0=Simulink.data.evalinGlobal(bdroot,get_param(gcb,'if0'));
      |   iksi=Simulink.data.evalinGlobal(bdroot,get_param(gcb,'iksi'));
      |   mechspeed=Simulink.data.evalinGlobal(bdroot,get_param(gcb,'mechspeed'));
      |   polepairs=Simulink.data.evalinGlobal(bdroot,get_param(gcb,'polepairs'));
      |   ADCMaxError=Simulink.data.evalinGlobal(bdroot,get_param(gcb,'ADCMaxError'));
      |   uscale=Simulink.data.evalinGlobal(bdroot,get_param(gcb,'uscale'));
      |   if (if0<=0)
      |     warning('Natural frequency f0 must be positive.');
      |   end
      |   if (iksi<=0)
      |     warning('Feedback loop attenuation must be positive.');
      |   end
      |   if (iksi>1)
      |     warning('Feedback loop attenuation must not exceed 1.');
      |   end
      |   if (mechspeed<=0)
      |     warning('Max. speed must be positive.');
      |   end
      |   if (polepairs<1)
      |     warning('Number of pole pairs must be a natural number (1, 2, 3, ...).');
      |   end
      |   if (round(polepairs)~=polepairs)
      |     warning('Number of pole pairs must be a natural number (1, 2, 3, ...).');
      |   end
      |   if (ADCMaxError<=0)
      |     warning('f32ADCMaxError must be positive.');
      |   end
      |   adcsc=ADCMaxError/uscale;
      |   f32ADCMaxError=round(adcsc*2^31);
      |   if f32ADCMaxError>2^31-1
      |     f32ADCMaxError=2^31-1;
      |     warning(['Parameter f32ADCMaxError of ' gcb ' exceeds the fixed-point range.']);
      |   end
      |   if f32ADCMaxError<-2^31
      |     f32ADCMaxError=-2^31;
      |     warning(['Parameter f32ADCMaxError of ' gcb ' exceeds the fixed-point range.']);
      |   end
      |   pgain=12.56637061435917*iksi*if0;
      |   igain=39.47841760435743*if0*if0;
      |   cc1=pgain+igain*SampleTime*0.5;
      |   cc2=-pgain+igain*SampleTime*0.5;
      |   wmax=polepairs*mechspeed*0.1047197551196598;
      |   cc1f=cc1*3.141592653589793/wmax;
      |   cc2f=cc2*3.141592653589793/wmax;
      |   u16NShiftPI=ceil(log2(abs(cc1f)));
      |   tmpsh=ceil(log2(abs(cc2f)));
      |   if u16NShiftPI<tmpsh
      |     u16NShiftPI=tmpsh;
      |   end
      |   if u16NShiftPI<0
      |     u16NShiftPI=0;
      |   end
      |   if u16NShiftPI>31
      |     u16NShiftPI=31;
      |     warning(['Parameter u16NShiftPI of ' gcb ' exceeds the fixed-point range.']);
      |   end
      |   f32CC1sc=round(cc1f*2^(-u16NShiftPI)*2^31);
      |   if f32CC1sc>2^31-1
      |     f32CC1sc=2^31-1;
      |     warning(['Parameter f32CC1sc of ' gcb ' exceeds the fixed-point range.']);
      |   end
      |   if f32CC1sc<-2^31
      |     f32CC1sc=-2^31;
      |     warning(['Parameter f32CC1sc of ' gcb ' exceeds the fixed-point range.']);
      |   end
      |   f32CC2sc=round(cc2f*2^(-u16NShiftPI)*2^31);
      |   if f32CC2sc>2^31-1
      |     f32CC2sc=2^31-1;
      |     warning(['Parameter f32CC2sc of ' gcb ' exceeds the fixed-point range.']);
      |   end
      |   if f32CC2sc<-2^31
      |     f32CC2sc=-2^31;
      |     warning(['Parameter f32CC2sc of ' gcb ' exceeds the fixed-point range.']);
      |   end
      |   f32LowerLimit=-2147483648;
      |   f32UpperLimit=2147483647;
      |   c1f=SampleTime*0.5*wmax/3.141592653589793;
      |   u16NShiftI=ceil(log2(abs(c1f)));
      |   if u16NShiftI<0
      |     u16NShiftI=0;
      |   end
      |   if u16NShiftI>31
      |     u16NShiftI=31;
      |     warning(['Parameter u16NShiftI of ' gcb ' exceeds the fixed-point range.']);
      |   end
      |   f32C1=round(c1f*2^(-u16NShiftI)*2^31);
      |   if f32C1>2^31-1
      |     f32C1=2^31-1;
      |     warning(['Parameter f32C1 of ' gcb ' exceeds the fixed-point range.']);
      |   end
      |   if f32C1<-2^31
      |     f32C1=-2^31;
      |     warning(['Parameter f32C1 of ' gcb ' exceeds the fixed-point range.']);
      |   end
      |   if isnan(f32ADCMaxError)
      |     if ~strcmp(f32ADCMaxError_bkup,'0')
      |       set_param(gcb,'f32ADCMaxError','0');
      |     end
      |   else
      |     tmps=num2str(f32ADCMaxError);
      |     if ~strcmp(f32ADCMaxError_bkup,tmps)
      |       set_param(gcb,'f32ADCMaxError',tmps);
      |     end
      |   end
      |   if isnan(f32CC1sc)
      |     if ~strcmp(f32CC1sc_bkup,'0')
      |       set_param(gcb,'f32CC1sc','0');
      |     end
      |   else
      |     tmps=num2str(f32CC1sc);
      |     if ~strcmp(f32CC1sc_bkup,tmps)
      |       set_param(gcb,'f32CC1sc',tmps);
      |     end
      |   end
      |   if isnan(f32CC2sc)
      |     if ~strcmp(f32CC2sc_bkup,'0')
      |       set_param(gcb,'f32CC2sc','0');
      |     end
      |   else
      |     tmps=num2str(f32CC2sc);
      |     if ~strcmp(f32CC2sc_bkup,tmps)
      |       set_param(gcb,'f32CC2sc',tmps);
      |     end
      |   end
      |   if isnan(f32UpperLimit)
      |     if ~strcmp(f32UpperLimit_bkup,'0')
      |       set_param(gcb,'f32UpperLimit','0');
      |     end
      |   else
      |     tmps=num2str(f32UpperLimit);
      |     if ~strcmp(f32UpperLimit_bkup,tmps)
      |       set_param(gcb,'f32UpperLimit',tmps);
      |     end
      |   end
      |   if isnan(f32LowerLimit)
      |     if ~strcmp(f32LowerLimit_bkup,'0')
      |       set_param(gcb,'f32LowerLimit','0');
      |     end
      |   else
      |     tmps=num2str(f32LowerLimit);
      |     if ~strcmp(f32LowerLimit_bkup,tmps)
      |       set_param(gcb,'f32LowerLimit',tmps);
      |     end
      |   end
      |   if isnan(u16NShiftPI)
      |     if ~strcmp(u16NShiftPI_bkup,'0')
      |       set_param(gcb,'u16NShiftPI','0');
      |     end
      |   else
      |     tmps=num2str(u16NShiftPI);
      |     if ~strcmp(u16NShiftPI_bkup,tmps)
      |       set_param(gcb,'u16NShiftPI',tmps);
      |     end
      |   end
      |   if isnan(f32C1)
      |     if ~strcmp(f32C1_bkup,'0')
      |       set_param(gcb,'f32C1','0');
      |     end
      |   else
      |     tmps=num2str(f32C1);
      |     if ~strcmp(f32C1_bkup,tmps)
      |       set_param(gcb,'f32C1',tmps);
      |     end
      |   end
      |   if isnan(u16NShiftI)
      |     if ~strcmp(u16NShiftI_bkup,'0')
      |       set_param(gcb,'u16NShiftI','0');
      |     end
      |   else
      |     tmps=num2str(u16NShiftI);
      |     if ~strcmp(u16NShiftI_bkup,tmps)
      |       set_param(gcb,'u16NShiftI',tmps);
      |     end
      |   end
      | end
      mask Callback mechspeed:
      | autoCalcEn=get_param(gcb,'autoCalcEn');
      | if strcmp(autoCalcEn,'on')
      |   SampleTime=Simulink.data.evalinGlobal(bdroot,get_param(gcb,'SampleTime'));
      |   if (SampleTime==-1)
      |     SampleTime=str2double(get_param(gcb,'SampleTime_1'));
      |   end
      |   f32ADCMaxError_bkup=get_param(gcb,'f32ADCMaxError');
      |   f32CC1sc_bkup=get_param(gcb,'f32CC1sc');
      |   f32CC2sc_bkup=get_param(gcb,'f32CC2sc');
      |   f32UpperLimit_bkup=get_param(gcb,'f32UpperLimit');
      |   f32LowerLimit_bkup=get_param(gcb,'f32LowerLimit');
      |   u16NShiftPI_bkup=get_param(gcb,'u16NShiftPI');
      |   f32C1_bkup=get_param(gcb,'f32C1');
      |   u16NShiftI_bkup=get_param(gcb,'u16NShiftI');
      |   if0=Simulink.data.evalinGlobal(bdroot,get_param(gcb,'if0'));
      |   iksi=Simulink.data.evalinGlobal(bdroot,get_param(gcb,'iksi'));
      |   mechspeed=Simulink.data.evalinGlobal(bdroot,get_param(gcb,'mechspeed'));
      |   polepairs=Simulink.data.evalinGlobal(bdroot,get_param(gcb,'polepairs'));
      |   ADCMaxError=Simulink.data.evalinGlobal(bdroot,get_param(gcb,'ADCMaxError'));
      |   uscale=Simulink.data.evalinGlobal(bdroot,get_param(gcb,'uscale'));
      |   if (if0<=0)
      |     warning('Natural frequency f0 must be positive.');
      |   end
      |   if (iksi<=0)
      |     warning('Feedback loop attenuation must be positive.');
      |   end
      |   if (iksi>1)
      |     warning('Feedback loop attenuation must not exceed 1.');
      |   end
      |   if (mechspeed<=0)
      |     warning('Max. speed must be positive.');
      |   end
      |   if (polepairs<1)
      |     warning('Number of pole pairs must be a natural number (1, 2, 3, ...).');
      |   end
      |   if (round(polepairs)~=polepairs)
      |     warning('Number of pole pairs must be a natural number (1, 2, 3, ...).');
      |   end
      |   if (ADCMaxError<=0)
      |     warning('f32ADCMaxError must be positive.');
      |   end
      |   adcsc=ADCMaxError/uscale;
      |   f32ADCMaxError=round(adcsc*2^31);
      |   if f32ADCMaxError>2^31-1
      |     f32ADCMaxError=2^31-1;
      |     warning(['Parameter f32ADCMaxError of ' gcb ' exceeds the fixed-point range.']);
      |   end
      |   if f32ADCMaxError<-2^31
      |     f32ADCMaxError=-2^31;
      |     warning(['Parameter f32ADCMaxError of ' gcb ' exceeds the fixed-point range.']);
      |   end
      |   pgain=12.56637061435917*iksi*if0;
      |   igain=39.47841760435743*if0*if0;
      |   cc1=pgain+igain*SampleTime*0.5;
      |   cc2=-pgain+igain*SampleTime*0.5;
      |   wmax=polepairs*mechspeed*0.1047197551196598;
      |   cc1f=cc1*3.141592653589793/wmax;
      |   cc2f=cc2*3.141592653589793/wmax;
      |   u16NShiftPI=ceil(log2(abs(cc1f)));
      |   tmpsh=ceil(log2(abs(cc2f)));
      |   if u16NShiftPI<tmpsh
      |     u16NShiftPI=tmpsh;
      |   end
      |   if u16NShiftPI<0
      |     u16NShiftPI=0;
      |   end
      |   if u16NShiftPI>31
      |     u16NShiftPI=31;
      |     warning(['Parameter u16NShiftPI of ' gcb ' exceeds the fixed-point range.']);
      |   end
      |   f32CC1sc=round(cc1f*2^(-u16NShiftPI)*2^31);
      |   if f32CC1sc>2^31-1
      |     f32CC1sc=2^31-1;
      |     warning(['Parameter f32CC1sc of ' gcb ' exceeds the fixed-point range.']);
      |   end
      |   if f32CC1sc<-2^31
      |     f32CC1sc=-2^31;
      |     warning(['Parameter f32CC1sc of ' gcb ' exceeds the fixed-point range.']);
      |   end
      |   f32CC2sc=round(cc2f*2^(-u16NShiftPI)*2^31);
      |   if f32CC2sc>2^31-1
      |     f32CC2sc=2^31-1;
      |     warning(['Parameter f32CC2sc of ' gcb ' exceeds the fixed-point range.']);
      |   end
      |   if f32CC2sc<-2^31
      |     f32CC2sc=-2^31;
      |     warning(['Parameter f32CC2sc of ' gcb ' exceeds the fixed-point range.']);
      |   end
      |   f32LowerLimit=-2147483648;
      |   f32UpperLimit=2147483647;
      |   c1f=SampleTime*0.5*wmax/3.141592653589793;
      |   u16NShiftI=ceil(log2(abs(c1f)));
      |   if u16NShiftI<0
      |     u16NShiftI=0;
      |   end
      |   if u16NShiftI>31
      |     u16NShiftI=31;
      |     warning(['Parameter u16NShiftI of ' gcb ' exceeds the fixed-point range.']);
      |   end
      |   f32C1=round(c1f*2^(-u16NShiftI)*2^31);
      |   if f32C1>2^31-1
      |     f32C1=2^31-1;
      |     warning(['Parameter f32C1 of ' gcb ' exceeds the fixed-point range.']);
      |   end
      |   if f32C1<-2^31
      |     f32C1=-2^31;
      |     warning(['Parameter f32C1 of ' gcb ' exceeds the fixed-point range.']);
      |   end
      |   if isnan(f32ADCMaxError)
      |     if ~strcmp(f32ADCMaxError_bkup,'0')
      |       set_param(gcb,'f32ADCMaxError','0');
      |     end
      |   else
      |     tmps=num2str(f32ADCMaxError);
      |     if ~strcmp(f32ADCMaxError_bkup,tmps)
      |       set_param(gcb,'f32ADCMaxError',tmps);
      |     end
      |   end
      |   if isnan(f32CC1sc)
      |     if ~strcmp(f32CC1sc_bkup,'0')
      |       set_param(gcb,'f32CC1sc','0');
      |     end
      |   else
      |     tmps=num2str(f32CC1sc);
      |     if ~strcmp(f32CC1sc_bkup,tmps)
      |       set_param(gcb,'f32CC1sc',tmps);
      |     end
      |   end
      |   if isnan(f32CC2sc)
      |     if ~strcmp(f32CC2sc_bkup,'0')
      |       set_param(gcb,'f32CC2sc','0');
      |     end
      |   else
      |     tmps=num2str(f32CC2sc);
      |     if ~strcmp(f32CC2sc_bkup,tmps)
      |       set_param(gcb,'f32CC2sc',tmps);
      |     end
      |   end
      |   if isnan(f32UpperLimit)
      |     if ~strcmp(f32UpperLimit_bkup,'0')
      |       set_param(gcb,'f32UpperLimit','0');
      |     end
      |   else
      |     tmps=num2str(f32UpperLimit);
      |     if ~strcmp(f32UpperLimit_bkup,tmps)
      |       set_param(gcb,'f32UpperLimit',tmps);
      |     end
      |   end
      |   if isnan(f32LowerLimit)
      |     if ~strcmp(f32LowerLimit_bkup,'0')
      |       set_param(gcb,'f32LowerLimit','0');
      |     end
      |   else
      |     tmps=num2str(f32LowerLimit);
      |     if ~strcmp(f32LowerLimit_bkup,tmps)
      |       set_param(gcb,'f32LowerLimit',tmps);
      |     end
      |   end
      |   if isnan(u16NShiftPI)
      |     if ~strcmp(u16NShiftPI_bkup,'0')
      |       set_param(gcb,'u16NShiftPI','0');
      |     end
      |   else
      |     tmps=num2str(u16NShiftPI);
      |     if ~strcmp(u16NShiftPI_bkup,tmps)
      |       set_param(gcb,'u16NShiftPI',tmps);
      |     end
      |   end
      |   if isnan(f32C1)
      |     if ~strcmp(f32C1_bkup,'0')
      |       set_param(gcb,'f32C1','0');
      |     end
      |   else
      |     tmps=num2str(f32C1);
      |     if ~strcmp(f32C1_bkup,tmps)
      |       set_param(gcb,'f32C1',tmps);
      |     end
      |   end
      |   if isnan(u16NShiftI)
      |     if ~strcmp(u16NShiftI_bkup,'0')
      |       set_param(gcb,'u16NShiftI','0');
      |     end
      |   else
      |     tmps=num2str(u16NShiftI);
      |     if ~strcmp(u16NShiftI_bkup,tmps)
      |       set_param(gcb,'u16NShiftI',tmps);
      |     end
      |   end
      | end
      mask Callback polepairs:
      | autoCalcEn=get_param(gcb,'autoCalcEn');
      | if strcmp(autoCalcEn,'on')
      |   SampleTime=Simulink.data.evalinGlobal(bdroot,get_param(gcb,'SampleTime'));
      |   if (SampleTime==-1)
      |     SampleTime=str2double(get_param(gcb,'SampleTime_1'));
      |   end
      |   f32ADCMaxError_bkup=get_param(gcb,'f32ADCMaxError');
      |   f32CC1sc_bkup=get_param(gcb,'f32CC1sc');
      |   f32CC2sc_bkup=get_param(gcb,'f32CC2sc');
      |   f32UpperLimit_bkup=get_param(gcb,'f32UpperLimit');
      |   f32LowerLimit_bkup=get_param(gcb,'f32LowerLimit');
      |   u16NShiftPI_bkup=get_param(gcb,'u16NShiftPI');
      |   f32C1_bkup=get_param(gcb,'f32C1');
      |   u16NShiftI_bkup=get_param(gcb,'u16NShiftI');
      |   if0=Simulink.data.evalinGlobal(bdroot,get_param(gcb,'if0'));
      |   iksi=Simulink.data.evalinGlobal(bdroot,get_param(gcb,'iksi'));
      |   mechspeed=Simulink.data.evalinGlobal(bdroot,get_param(gcb,'mechspeed'));
      |   polepairs=Simulink.data.evalinGlobal(bdroot,get_param(gcb,'polepairs'));
      |   ADCMaxError=Simulink.data.evalinGlobal(bdroot,get_param(gcb,'ADCMaxError'));
      |   uscale=Simulink.data.evalinGlobal(bdroot,get_param(gcb,'uscale'));
      |   if (if0<=0)
      |     warning('Natural frequency f0 must be positive.');
      |   end
      |   if (iksi<=0)
      |     warning('Feedback loop attenuation must be positive.');
      |   end
      |   if (iksi>1)
      |     warning('Feedback loop attenuation must not exceed 1.');
      |   end
      |   if (mechspeed<=0)
      |     warning('Max. speed must be positive.');
      |   end
      |   if (polepairs<1)
      |     warning('Number of pole pairs must be a natural number (1, 2, 3, ...).');
      |   end
      |   if (round(polepairs)~=polepairs)
      |     warning('Number of pole pairs must be a natural number (1, 2, 3, ...).');
      |   end
      |   if (ADCMaxError<=0)
      |     warning('f32ADCMaxError must be positive.');
      |   end
      |   adcsc=ADCMaxError/uscale;
      |   f32ADCMaxError=round(adcsc*2^31);
      |   if f32ADCMaxError>2^31-1
      |     f32ADCMaxError=2^31-1;
      |     warning(['Parameter f32ADCMaxError of ' gcb ' exceeds the fixed-point range.']);
      |   end
      |   if f32ADCMaxError<-2^31
      |     f32ADCMaxError=-2^31;
      |     warning(['Parameter f32ADCMaxError of ' gcb ' exceeds the fixed-point range.']);
      |   end
      |   pgain=12.56637061435917*iksi*if0;
      |   igain=39.47841760435743*if0*if0;
      |   cc1=pgain+igain*SampleTime*0.5;
      |   cc2=-pgain+igain*SampleTime*0.5;
      |   wmax=polepairs*mechspeed*0.1047197551196598;
      |   cc1f=cc1*3.141592653589793/wmax;
      |   cc2f=cc2*3.141592653589793/wmax;
      |   u16NShiftPI=ceil(log2(abs(cc1f)));
      |   tmpsh=ceil(log2(abs(cc2f)));
      |   if u16NShiftPI<tmpsh
      |     u16NShiftPI=tmpsh;
      |   end
      |   if u16NShiftPI<0
      |     u16NShiftPI=0;
      |   end
      |   if u16NShiftPI>31
      |     u16NShiftPI=31;
      |     warning(['Parameter u16NShiftPI of ' gcb ' exceeds the fixed-point range.']);
      |   end
      |   f32CC1sc=round(cc1f*2^(-u16NShiftPI)*2^31);
      |   if f32CC1sc>2^31-1
      |     f32CC1sc=2^31-1;
      |     warning(['Parameter f32CC1sc of ' gcb ' exceeds the fixed-point range.']);
      |   end
      |   if f32CC1sc<-2^31
      |     f32CC1sc=-2^31;
      |     warning(['Parameter f32CC1sc of ' gcb ' exceeds the fixed-point range.']);
      |   end
      |   f32CC2sc=round(cc2f*2^(-u16NShiftPI)*2^31);
      |   if f32CC2sc>2^31-1
      |     f32CC2sc=2^31-1;
      |     warning(['Parameter f32CC2sc of ' gcb ' exceeds the fixed-point range.']);
      |   end
      |   if f32CC2sc<-2^31
      |     f32CC2sc=-2^31;
      |     warning(['Parameter f32CC2sc of ' gcb ' exceeds the fixed-point range.']);
      |   end
      |   f32LowerLimit=-2147483648;
      |   f32UpperLimit=2147483647;
      |   c1f=SampleTime*0.5*wmax/3.141592653589793;
      |   u16NShiftI=ceil(log2(abs(c1f)));
      |   if u16NShiftI<0
      |     u16NShiftI=0;
      |   end
      |   if u16NShiftI>31
      |     u16NShiftI=31;
      |     warning(['Parameter u16NShiftI of ' gcb ' exceeds the fixed-point range.']);
      |   end
      |   f32C1=round(c1f*2^(-u16NShiftI)*2^31);
      |   if f32C1>2^31-1
      |     f32C1=2^31-1;
      |     warning(['Parameter f32C1 of ' gcb ' exceeds the fixed-point range.']);
      |   end
      |   if f32C1<-2^31
      |     f32C1=-2^31;
      |     warning(['Parameter f32C1 of ' gcb ' exceeds the fixed-point range.']);
      |   end
      |   if isnan(f32ADCMaxError)
      |     if ~strcmp(f32ADCMaxError_bkup,'0')
      |       set_param(gcb,'f32ADCMaxError','0');
      |     end
      |   else
      |     tmps=num2str(f32ADCMaxError);
      |     if ~strcmp(f32ADCMaxError_bkup,tmps)
      |       set_param(gcb,'f32ADCMaxError',tmps);
      |     end
      |   end
      |   if isnan(f32CC1sc)
      |     if ~strcmp(f32CC1sc_bkup,'0')
      |       set_param(gcb,'f32CC1sc','0');
      |     end
      |   else
      |     tmps=num2str(f32CC1sc);
      |     if ~strcmp(f32CC1sc_bkup,tmps)
      |       set_param(gcb,'f32CC1sc',tmps);
      |     end
      |   end
      |   if isnan(f32CC2sc)
      |     if ~strcmp(f32CC2sc_bkup,'0')
      |       set_param(gcb,'f32CC2sc','0');
      |     end
      |   else
      |     tmps=num2str(f32CC2sc);
      |     if ~strcmp(f32CC2sc_bkup,tmps)
      |       set_param(gcb,'f32CC2sc',tmps);
      |     end
      |   end
      |   if isnan(f32UpperLimit)
      |     if ~strcmp(f32UpperLimit_bkup,'0')
      |       set_param(gcb,'f32UpperLimit','0');
      |     end
      |   else
      |     tmps=num2str(f32UpperLimit);
      |     if ~strcmp(f32UpperLimit_bkup,tmps)
      |       set_param(gcb,'f32UpperLimit',tmps);
      |     end
      |   end
      |   if isnan(f32LowerLimit)
      |     if ~strcmp(f32LowerLimit_bkup,'0')
      |       set_param(gcb,'f32LowerLimit','0');
      |     end
      |   else
      |     tmps=num2str(f32LowerLimit);
      |     if ~strcmp(f32LowerLimit_bkup,tmps)
      |       set_param(gcb,'f32LowerLimit',tmps);
      |     end
      |   end
      |   if isnan(u16NShiftPI)
      |     if ~strcmp(u16NShiftPI_bkup,'0')
      |       set_param(gcb,'u16NShiftPI','0');
      |     end
      |   else
      |     tmps=num2str(u16NShiftPI);
      |     if ~strcmp(u16NShiftPI_bkup,tmps)
      |       set_param(gcb,'u16NShiftPI',tmps);
      |     end
      |   end
      |   if isnan(f32C1)
      |     if ~strcmp(f32C1_bkup,'0')
      |       set_param(gcb,'f32C1','0');
      |     end
      |   else
      |     tmps=num2str(f32C1);
      |     if ~strcmp(f32C1_bkup,tmps)
      |       set_param(gcb,'f32C1',tmps);
      |     end
      |   end
      |   if isnan(u16NShiftI)
      |     if ~strcmp(u16NShiftI_bkup,'0')
      |       set_param(gcb,'u16NShiftI','0');
      |     end
      |   else
      |     tmps=num2str(u16NShiftI);
      |     if ~strcmp(u16NShiftI_bkup,tmps)
      |       set_param(gcb,'u16NShiftI',tmps);
      |     end
      |   end
      | end
      mask Callback ADCMaxError:
      | autoCalcEn=get_param(gcb,'autoCalcEn');
      | if strcmp(autoCalcEn,'on')
      |   SampleTime=Simulink.data.evalinGlobal(bdroot,get_param(gcb,'SampleTime'));
      |   if (SampleTime==-1)
      |     SampleTime=str2double(get_param(gcb,'SampleTime_1'));
      |   end
      |   f32ADCMaxError_bkup=get_param(gcb,'f32ADCMaxError');
      |   f32CC1sc_bkup=get_param(gcb,'f32CC1sc');
      |   f32CC2sc_bkup=get_param(gcb,'f32CC2sc');
      |   f32UpperLimit_bkup=get_param(gcb,'f32UpperLimit');
      |   f32LowerLimit_bkup=get_param(gcb,'f32LowerLimit');
      |   u16NShiftPI_bkup=get_param(gcb,'u16NShiftPI');
      |   f32C1_bkup=get_param(gcb,'f32C1');
      |   u16NShiftI_bkup=get_param(gcb,'u16NShiftI');
      |   if0=Simulink.data.evalinGlobal(bdroot,get_param(gcb,'if0'));
      |   iksi=Simulink.data.evalinGlobal(bdroot,get_param(gcb,'iksi'));
      |   mechspeed=Simulink.data.evalinGlobal(bdroot,get_param(gcb,'mechspeed'));
      |   polepairs=Simulink.data.evalinGlobal(bdroot,get_param(gcb,'polepairs'));
      |   ADCMaxError=Simulink.data.evalinGlobal(bdroot,get_param(gcb,'ADCMaxError'));
      |   uscale=Simulink.data.evalinGlobal(bdroot,get_param(gcb,'uscale'));
      |   if (if0<=0)
      |     warning('Natural frequency f0 must be positive.');
      |   end
      |   if (iksi<=0)
      |     warning('Feedback loop attenuation must be positive.');
      |   end
      |   if (iksi>1)
      |     warning('Feedback loop attenuation must not exceed 1.');
      |   end
      |   if (mechspeed<=0)
      |     warning('Max. speed must be positive.');
      |   end
      |   if (polepairs<1)
      |     warning('Number of pole pairs must be a natural number (1, 2, 3, ...).');
      |   end
      |   if (round(polepairs)~=polepairs)
      |     warning('Number of pole pairs must be a natural number (1, 2, 3, ...).');
      |   end
      |   if (ADCMaxError<=0)
      |     warning('f32ADCMaxError must be positive.');
      |   end
      |   adcsc=ADCMaxError/uscale;
      |   f32ADCMaxError=round(adcsc*2^31);
      |   if f32ADCMaxError>2^31-1
      |     f32ADCMaxError=2^31-1;
      |     warning(['Parameter f32ADCMaxError of ' gcb ' exceeds the fixed-point range.']);
      |   end
      |   if f32ADCMaxError<-2^31
      |     f32ADCMaxError=-2^31;
      |     warning(['Parameter f32ADCMaxError of ' gcb ' exceeds the fixed-point range.']);
      |   end
      |   pgain=12.56637061435917*iksi*if0;
      |   igain=39.47841760435743*if0*if0;
      |   cc1=pgain+igain*SampleTime*0.5;
      |   cc2=-pgain+igain*SampleTime*0.5;
      |   wmax=polepairs*mechspeed*0.1047197551196598;
      |   cc1f=cc1*3.141592653589793/wmax;
      |   cc2f=cc2*3.141592653589793/wmax;
      |   u16NShiftPI=ceil(log2(abs(cc1f)));
      |   tmpsh=ceil(log2(abs(cc2f)));
      |   if u16NShiftPI<tmpsh
      |     u16NShiftPI=tmpsh;
      |   end
      |   if u16NShiftPI<0
      |     u16NShiftPI=0;
      |   end
      |   if u16NShiftPI>31
      |     u16NShiftPI=31;
      |     warning(['Parameter u16NShiftPI of ' gcb ' exceeds the fixed-point range.']);
      |   end
      |   f32CC1sc=round(cc1f*2^(-u16NShiftPI)*2^31);
      |   if f32CC1sc>2^31-1
      |     f32CC1sc=2^31-1;
      |     warning(['Parameter f32CC1sc of ' gcb ' exceeds the fixed-point range.']);
      |   end
      |   if f32CC1sc<-2^31
      |     f32CC1sc=-2^31;
      |     warning(['Parameter f32CC1sc of ' gcb ' exceeds the fixed-point range.']);
      |   end
      |   f32CC2sc=round(cc2f*2^(-u16NShiftPI)*2^31);
      |   if f32CC2sc>2^31-1
      |     f32CC2sc=2^31-1;
      |     warning(['Parameter f32CC2sc of ' gcb ' exceeds the fixed-point range.']);
      |   end
      |   if f32CC2sc<-2^31
      |     f32CC2sc=-2^31;
      |     warning(['Parameter f32CC2sc of ' gcb ' exceeds the fixed-point range.']);
      |   end
      |   f32LowerLimit=-2147483648;
      |   f32UpperLimit=2147483647;
      |   c1f=SampleTime*0.5*wmax/3.141592653589793;
      |   u16NShiftI=ceil(log2(abs(c1f)));
      |   if u16NShiftI<0
      |     u16NShiftI=0;
      |   end
      |   if u16NShiftI>31
      |     u16NShiftI=31;
      |     warning(['Parameter u16NShiftI of ' gcb ' exceeds the fixed-point range.']);
      |   end
      |   f32C1=round(c1f*2^(-u16NShiftI)*2^31);
      |   if f32C1>2^31-1
      |     f32C1=2^31-1;
      |     warning(['Parameter f32C1 of ' gcb ' exceeds the fixed-point range.']);
      |   end
      |   if f32C1<-2^31
      |     f32C1=-2^31;
      |     warning(['Parameter f32C1 of ' gcb ' exceeds the fixed-point range.']);
      |   end
      |   if isnan(f32ADCMaxError)
      |     if ~strcmp(f32ADCMaxError_bkup,'0')
      |       set_param(gcb,'f32ADCMaxError','0');
      |     end
      |   else
      |     tmps=num2str(f32ADCMaxError);
      |     if ~strcmp(f32ADCMaxError_bkup,tmps)
      |       set_param(gcb,'f32ADCMaxError',tmps);
      |     end
      |   end
      |   if isnan(f32CC1sc)
      |     if ~strcmp(f32CC1sc_bkup,'0')
      |       set_param(gcb,'f32CC1sc','0');
      |     end
      |   else
      |     tmps=num2str(f32CC1sc);
      |     if ~strcmp(f32CC1sc_bkup,tmps)
      |       set_param(gcb,'f32CC1sc',tmps);
      |     end
      |   end
      |   if isnan(f32CC2sc)
      |     if ~strcmp(f32CC2sc_bkup,'0')
      |       set_param(gcb,'f32CC2sc','0');
      |     end
      |   else
      |     tmps=num2str(f32CC2sc);
      |     if ~strcmp(f32CC2sc_bkup,tmps)
      |       set_param(gcb,'f32CC2sc',tmps);
      |     end
      |   end
      |   if isnan(f32UpperLimit)
      |     if ~strcmp(f32UpperLimit_bkup,'0')
      |       set_param(gcb,'f32UpperLimit','0');
      |     end
      |   else
      |     tmps=num2str(f32UpperLimit);
      |     if ~strcmp(f32UpperLimit_bkup,tmps)
      |       set_param(gcb,'f32UpperLimit',tmps);
      |     end
      |   end
      |   if isnan(f32LowerLimit)
      |     if ~strcmp(f32LowerLimit_bkup,'0')
      |       set_param(gcb,'f32LowerLimit','0');
      |     end
      |   else
      |     tmps=num2str(f32LowerLimit);
      |     if ~strcmp(f32LowerLimit_bkup,tmps)
      |       set_param(gcb,'f32LowerLimit',tmps);
      |     end
      |   end
      |   if isnan(u16NShiftPI)
      |     if ~strcmp(u16NShiftPI_bkup,'0')
      |       set_param(gcb,'u16NShiftPI','0');
      |     end
      |   else
      |     tmps=num2str(u16NShiftPI);
      |     if ~strcmp(u16NShiftPI_bkup,tmps)
      |       set_param(gcb,'u16NShiftPI',tmps);
      |     end
      |   end
      |   if isnan(f32C1)
      |     if ~strcmp(f32C1_bkup,'0')
      |       set_param(gcb,'f32C1','0');
      |     end
      |   else
      |     tmps=num2str(f32C1);
      |     if ~strcmp(f32C1_bkup,tmps)
      |       set_param(gcb,'f32C1',tmps);
      |     end
      |   end
      |   if isnan(u16NShiftI)
      |     if ~strcmp(u16NShiftI_bkup,'0')
      |       set_param(gcb,'u16NShiftI','0');
      |     end
      |   else
      |     tmps=num2str(u16NShiftI);
      |     if ~strcmp(u16NShiftI_bkup,tmps)
      |       set_param(gcb,'u16NShiftI',tmps);
      |     end
      |   end
      | end
      mask Callback uscale:
      | autoCalcEn=get_param(gcb,'autoCalcEn');
      | if strcmp(autoCalcEn,'on')
      |   SampleTime=Simulink.data.evalinGlobal(bdroot,get_param(gcb,'SampleTime'));
      |   if (SampleTime==-1)
      |     SampleTime=str2double(get_param(gcb,'SampleTime_1'));
      |   end
      |   f32ADCMaxError_bkup=get_param(gcb,'f32ADCMaxError');
      |   f32CC1sc_bkup=get_param(gcb,'f32CC1sc');
      |   f32CC2sc_bkup=get_param(gcb,'f32CC2sc');
      |   f32UpperLimit_bkup=get_param(gcb,'f32UpperLimit');
      |   f32LowerLimit_bkup=get_param(gcb,'f32LowerLimit');
      |   u16NShiftPI_bkup=get_param(gcb,'u16NShiftPI');
      |   f32C1_bkup=get_param(gcb,'f32C1');
      |   u16NShiftI_bkup=get_param(gcb,'u16NShiftI');
      |   if0=Simulink.data.evalinGlobal(bdroot,get_param(gcb,'if0'));
      |   iksi=Simulink.data.evalinGlobal(bdroot,get_param(gcb,'iksi'));
      |   mechspeed=Simulink.data.evalinGlobal(bdroot,get_param(gcb,'mechspeed'));
      |   polepairs=Simulink.data.evalinGlobal(bdroot,get_param(gcb,'polepairs'));
      |   ADCMaxError=Simulink.data.evalinGlobal(bdroot,get_param(gcb,'ADCMaxError'));
      |   uscale=Simulink.data.evalinGlobal(bdroot,get_param(gcb,'uscale'));
      |   if (if0<=0)
      |     warning('Natural frequency f0 must be positive.');
      |   end
      |   if (iksi<=0)
      |     warning('Feedback loop attenuation must be positive.');
      |   end
      |   if (iksi>1)
      |     warning('Feedback loop attenuation must not exceed 1.');
      |   end
      |   if (mechspeed<=0)
      |     warning('Max. speed must be positive.');
      |   end
      |   if (polepairs<1)
      |     warning('Number of pole pairs must be a natural number (1, 2, 3, ...).');
      |   end
      |   if (round(polepairs)~=polepairs)
      |     warning('Number of pole pairs must be a natural number (1, 2, 3, ...).');
      |   end
      |   if (ADCMaxError<=0)
      |     warning('f32ADCMaxError must be positive.');
      |   end
      |   adcsc=ADCMaxError/uscale;
      |   f32ADCMaxError=round(adcsc*2^31);
      |   if f32ADCMaxError>2^31-1
      |     f32ADCMaxError=2^31-1;
      |     warning(['Parameter f32ADCMaxError of ' gcb ' exceeds the fixed-point range.']);
      |   end
      |   if f32ADCMaxError<-2^31
      |     f32ADCMaxError=-2^31;
      |     warning(['Parameter f32ADCMaxError of ' gcb ' exceeds the fixed-point range.']);
      |   end
      |   pgain=12.56637061435917*iksi*if0;
      |   igain=39.47841760435743*if0*if0;
      |   cc1=pgain+igain*SampleTime*0.5;
      |   cc2=-pgain+igain*SampleTime*0.5;
      |   wmax=polepairs*mechspeed*0.1047197551196598;
      |   cc1f=cc1*3.141592653589793/wmax;
      |   cc2f=cc2*3.141592653589793/wmax;
      |   u16NShiftPI=ceil(log2(abs(cc1f)));
      |   tmpsh=ceil(log2(abs(cc2f)));
      |   if u16NShiftPI<tmpsh
      |     u16NShiftPI=tmpsh;
      |   end
      |   if u16NShiftPI<0
      |     u16NShiftPI=0;
      |   end
      |   if u16NShiftPI>31
      |     u16NShiftPI=31;
      |     warning(['Parameter u16NShiftPI of ' gcb ' exceeds the fixed-point range.']);
      |   end
      |   f32CC1sc=round(cc1f*2^(-u16NShiftPI)*2^31);
      |   if f32CC1sc>2^31-1
      |     f32CC1sc=2^31-1;
      |     warning(['Parameter f32CC1sc of ' gcb ' exceeds the fixed-point range.']);
      |   end
      |   if f32CC1sc<-2^31
      |     f32CC1sc=-2^31;
      |     warning(['Parameter f32CC1sc of ' gcb ' exceeds the fixed-point range.']);
      |   end
      |   f32CC2sc=round(cc2f*2^(-u16NShiftPI)*2^31);
      |   if f32CC2sc>2^31-1
      |     f32CC2sc=2^31-1;
      |     warning(['Parameter f32CC2sc of ' gcb ' exceeds the fixed-point range.']);
      |   end
      |   if f32CC2sc<-2^31
      |     f32CC2sc=-2^31;
      |     warning(['Parameter f32CC2sc of ' gcb ' exceeds the fixed-point range.']);
      |   end
      |   f32LowerLimit=-2147483648;
      |   f32UpperLimit=2147483647;
      |   c1f=SampleTime*0.5*wmax/3.141592653589793;
      |   u16NShiftI=ceil(log2(abs(c1f)));
      |   if u16NShiftI<0
      |     u16NShiftI=0;
      |   end
      |   if u16NShiftI>31
      |     u16NShiftI=31;
      |     warning(['Parameter u16NShiftI of ' gcb ' exceeds the fixed-point range.']);
      |   end
      |   f32C1=round(c1f*2^(-u16NShiftI)*2^31);
      |   if f32C1>2^31-1
      |     f32C1=2^31-1;
      |     warning(['Parameter f32C1 of ' gcb ' exceeds the fixed-point range.']);
      |   end
      |   if f32C1<-2^31
      |     f32C1=-2^31;
      |     warning(['Parameter f32C1 of ' gcb ' exceeds the fixed-point range.']);
      |   end
      |   if isnan(f32ADCMaxError)
      |     if ~strcmp(f32ADCMaxError_bkup,'0')
      |       set_param(gcb,'f32ADCMaxError','0');
      |     end
      |   else
      |     tmps=num2str(f32ADCMaxError);
      |     if ~strcmp(f32ADCMaxError_bkup,tmps)
      |       set_param(gcb,'f32ADCMaxError',tmps);
      |     end
      |   end
      |   if isnan(f32CC1sc)
      |     if ~strcmp(f32CC1sc_bkup,'0')
      |       set_param(gcb,'f32CC1sc','0');
      |     end
      |   else
      |     tmps=num2str(f32CC1sc);
      |     if ~strcmp(f32CC1sc_bkup,tmps)
      |       set_param(gcb,'f32CC1sc',tmps);
      |     end
      |   end
      |   if isnan(f32CC2sc)
      |     if ~strcmp(f32CC2sc_bkup,'0')
      |       set_param(gcb,'f32CC2sc','0');
      |     end
      |   else
      |     tmps=num2str(f32CC2sc);
      |     if ~strcmp(f32CC2sc_bkup,tmps)
      |       set_param(gcb,'f32CC2sc',tmps);
      |     end
      |   end
      |   if isnan(f32UpperLimit)
      |     if ~strcmp(f32UpperLimit_bkup,'0')
      |       set_param(gcb,'f32UpperLimit','0');
      |     end
      |   else
      |     tmps=num2str(f32UpperLimit);
      |     if ~strcmp(f32UpperLimit_bkup,tmps)
      |       set_param(gcb,'f32UpperLimit',tmps);
      |     end
      |   end
      |   if isnan(f32LowerLimit)
      |     if ~strcmp(f32LowerLimit_bkup,'0')
      |       set_param(gcb,'f32LowerLimit','0');
      |     end
      |   else
      |     tmps=num2str(f32LowerLimit);
      |     if ~strcmp(f32LowerLimit_bkup,tmps)
      |       set_param(gcb,'f32LowerLimit',tmps);
      |     end
      |   end
      |   if isnan(u16NShiftPI)
      |     if ~strcmp(u16NShiftPI_bkup,'0')
      |       set_param(gcb,'u16NShiftPI','0');
      |     end
      |   else
      |     tmps=num2str(u16NShiftPI);
      |     if ~strcmp(u16NShiftPI_bkup,tmps)
      |       set_param(gcb,'u16NShiftPI',tmps);
      |     end
      |   end
      |   if isnan(f32C1)
      |     if ~strcmp(f32C1_bkup,'0')
      |       set_param(gcb,'f32C1','0');
      |     end
      |   else
      |     tmps=num2str(f32C1);
      |     if ~strcmp(f32C1_bkup,tmps)
      |       set_param(gcb,'f32C1',tmps);
      |     end
      |   end
      |   if isnan(u16NShiftI)
      |     if ~strcmp(u16NShiftI_bkup,'0')
      |       set_param(gcb,'u16NShiftI','0');
      |     end
      |   else
      |     tmps=num2str(u16NShiftI);
      |     if ~strcmp(u16NShiftI_bkup,tmps)
      |       set_param(gcb,'u16NShiftI',tmps);
      |     end
      |   end
      | end
      mask Callback autoCalcEn:
      | maskStr=get_param(gcb,'showStates');
      | if strcmp(maskStr,'Hide (faster execution)')
      |   p=Simulink.Mask.get(gcb);
      |   autoCalcEn=get_param(gcb,'autoCalcEn');
      |   hintText=p.getDialogControl('timeHint');
      |   if strcmp(autoCalcEn,'on')
      |     param=p.getParameter('uscale');
      |     if strcmp(param.Enabled,'off')
      |       SampleTime=Simulink.data.evalinGlobal(bdroot,get_param(gcb,'SampleTime'));
      |       if SampleTime==-1
      |         SampleTime=str2double(get_param(gcb,'SampleTime_1'));
      |         if isnan(SampleTime)
      |           hintText.Prompt=['Note: Implementation parameters cannot be calculated yet because the block''s inherited sample time is unknown. Simulink will update the sample time when you run the simulation.'];
      |         else
      |           hintText.Prompt=['Caution: Implementation parameters depend on inherited sample time. Make sure that the sample time of the block''s inputs corresponds to the sampling period in the target application.'];
      |         end
      |       else
      |         hintText.Prompt='Caution: Implementation parameters depend on the sample time. Make sure that the simulation time step corresponds to the sampling period in the target application.';
      |       end
      |       p=Simulink.Mask.get(gcb);
      |       param=p.getParameter('if0');
      |       param.set('Enabled','on');
      |       param=p.getParameter('iksi');
      |       param.set('Enabled','on');
      |       param=p.getParameter('mechspeed');
      |       param.set('Enabled','on');
      |       param=p.getParameter('polepairs');
      |       param.set('Enabled','on');
      |       param=p.getParameter('ADCMaxError');
      |       param.set('Enabled','on');
      |       param=p.getParameter('uscale');
      |       param.set('Enabled','on');
      |     else
      |       SampleTime=Simulink.data.evalinGlobal(bdroot,get_param(gcb,'SampleTime'));
      |       if SampleTime==-1
      |         SampleTime=str2double(get_param(gcb,'SampleTime_1'));
      |       end
      |     end
      |     f32ADCMaxError_bkup=get_param(gcb,'f32ADCMaxError');
      |     f32CC1sc_bkup=get_param(gcb,'f32CC1sc');
      |     f32CC2sc_bkup=get_param(gcb,'f32CC2sc');
      |     f32UpperLimit_bkup=get_param(gcb,'f32UpperLimit');
      |     f32LowerLimit_bkup=get_param(gcb,'f32LowerLimit');
      |     u16NShiftPI_bkup=get_param(gcb,'u16NShiftPI');
      |     f32C1_bkup=get_param(gcb,'f32C1');
      |     u16NShiftI_bkup=get_param(gcb,'u16NShiftI');
      |     if0=Simulink.data.evalinGlobal(bdroot,get_param(gcb,'if0'));
      |     iksi=Simulink.data.evalinGlobal(bdroot,get_param(gcb,'iksi'));
      |     mechspeed=Simulink.data.evalinGlobal(bdroot,get_param(gcb,'mechspeed'));
      |     polepairs=Simulink.data.evalinGlobal(bdroot,get_param(gcb,'polepairs'));
      |     ADCMaxError=Simulink.data.evalinGlobal(bdroot,get_param(gcb,'ADCMaxError'));
      |     uscale=Simulink.data.evalinGlobal(bdroot,get_param(gcb,'uscale'));
      |     if (if0<=0)
      |       warning('Natural frequency f0 must be positive.');
      |     end
      |     if (iksi<=0)
      |       warning('Feedback loop attenuation must be positive.');
      |     end
      |     if (iksi>1)
      |       warning('Feedback loop attenuation must not exceed 1.');
      |     end
      |     if (mechspeed<=0)
      |       warning('Max. speed must be positive.');
      |     end
      |     if (polepairs<1)
      |       warning('Number of pole pairs must be a natural number (1, 2, 3, ...).');
      |     end
      |     if (round(polepairs)~=polepairs)
      |       warning('Number of pole pairs must be a natural number (1, 2, 3, ...).');
      |     end
      |     if (ADCMaxError<=0)
      |       warning('f32ADCMaxError must be positive.');
      |     end
      |     adcsc=ADCMaxError/uscale;
      |     f32ADCMaxError=round(adcsc*2^31);
      |     if f32ADCMaxError>2^31-1
      |       f32ADCMaxError=2^31-1;
      |       warning(['Parameter f32ADCMaxError of ' gcb ' exceeds the fixed-point range.']);
      |     end
      |     if f32ADCMaxError<-2^31
      |       f32ADCMaxError=-2^31;
      |       warning(['Parameter f32ADCMaxError of ' gcb ' exceeds the fixed-point range.']);
      |     end
      |     pgain=12.56637061435917*iksi*if0;
      |     igain=39.47841760435743*if0*if0;
      |     cc1=pgain+igain*SampleTime*0.5;
      |     cc2=-pgain+igain*SampleTime*0.5;
      |     wmax=polepairs*mechspeed*0.1047197551196598;
      |     cc1f=cc1*3.141592653589793/wmax;
      |     cc2f=cc2*3.141592653589793/wmax;
      |     u16NShiftPI=ceil(log2(abs(cc1f)));
      |     tmpsh=ceil(log2(abs(cc2f)));
      |     if u16NShiftPI<tmpsh
      |       u16NShiftPI=tmpsh;
      |     end
      |     if u16NShiftPI<0
      |       u16NShiftPI=0;
      |     end
      |     if u16NShiftPI>31
      |       u16NShiftPI=31;
      |       warning(['Parameter u16NShiftPI of ' gcb ' exceeds the fixed-point range.']);
      |     end
      |     f32CC1sc=round(cc1f*2^(-u16NShiftPI)*2^31);
      |     if f32CC1sc>2^31-1
      |       f32CC1sc=2^31-1;
      |       warning(['Parameter f32CC1sc of ' gcb ' exceeds the fixed-point range.']);
      |     end
      |     if f32CC1sc<-2^31
      |       f32CC1sc=-2^31;
      |       warning(['Parameter f32CC1sc of ' gcb ' exceeds the fixed-point range.']);
      |     end
      |     f32CC2sc=round(cc2f*2^(-u16NShiftPI)*2^31);
      |     if f32CC2sc>2^31-1
      |       f32CC2sc=2^31-1;
      |       warning(['Parameter f32CC2sc of ' gcb ' exceeds the fixed-point range.']);
      |     end
      |     if f32CC2sc<-2^31
      |       f32CC2sc=-2^31;
      |       warning(['Parameter f32CC2sc of ' gcb ' exceeds the fixed-point range.']);
      |     end
      |     f32LowerLimit=-2147483648;
      |     f32UpperLimit=2147483647;
      |     c1f=SampleTime*0.5*wmax/3.141592653589793;
      |     u16NShiftI=ceil(log2(abs(c1f)));
      |     if u16NShiftI<0
      |       u16NShiftI=0;
      |     end
      |     if u16NShiftI>31
      |       u16NShiftI=31;
      |       warning(['Parameter u16NShiftI of ' gcb ' exceeds the fixed-point range.']);
      |     end
      |     f32C1=round(c1f*2^(-u16NShiftI)*2^31);
      |     if f32C1>2^31-1
      |       f32C1=2^31-1;
      |       warning(['Parameter f32C1 of ' gcb ' exceeds the fixed-point range.']);
      |     end
      |     if f32C1<-2^31
      |       f32C1=-2^31;
      |       warning(['Parameter f32C1 of ' gcb ' exceeds the fixed-point range.']);
      |     end
      |     if isnan(f32ADCMaxError)
      |       if ~strcmp(f32ADCMaxError_bkup,'0')
      |         set_param(gcb,'f32ADCMaxError','0');
      |       end
      |     else
      |       tmps=num2str(f32ADCMaxError);
      |       if ~strcmp(f32ADCMaxError_bkup,tmps)
      |         set_param(gcb,'f32ADCMaxError',tmps);
      |       end
      |     end
      |     if isnan(f32CC1sc)
      |       if ~strcmp(f32CC1sc_bkup,'0')
      |         set_param(gcb,'f32CC1sc','0');
      |       end
      |     else
      |       tmps=num2str(f32CC1sc);
      |       if ~strcmp(f32CC1sc_bkup,tmps)
      |         set_param(gcb,'f32CC1sc',tmps);
      |       end
      |     end
      |     if isnan(f32CC2sc)
      |       if ~strcmp(f32CC2sc_bkup,'0')
      |         set_param(gcb,'f32CC2sc','0');
      |       end
      |     else
      |       tmps=num2str(f32CC2sc);
      |       if ~strcmp(f32CC2sc_bkup,tmps)
      |         set_param(gcb,'f32CC2sc',tmps);
      |       end
      |     end
      |     if isnan(f32UpperLimit)
      |       if ~strcmp(f32UpperLimit_bkup,'0')
      |         set_param(gcb,'f32UpperLimit','0');
      |       end
      |     else
      |       tmps=num2str(f32UpperLimit);
      |       if ~strcmp(f32UpperLimit_bkup,tmps)
      |         set_param(gcb,'f32UpperLimit',tmps);
      |       end
      |     end
      |     if isnan(f32LowerLimit)
      |       if ~strcmp(f32LowerLimit_bkup,'0')
      |         set_param(gcb,'f32LowerLimit','0');
      |       end
      |     else
      |       tmps=num2str(f32LowerLimit);
      |       if ~strcmp(f32LowerLimit_bkup,tmps)
      |         set_param(gcb,'f32LowerLimit',tmps);
      |       end
      |     end
      |     if isnan(u16NShiftPI)
      |       if ~strcmp(u16NShiftPI_bkup,'0')
      |         set_param(gcb,'u16NShiftPI','0');
      |       end
      |     else
      |       tmps=num2str(u16NShiftPI);
      |       if ~strcmp(u16NShiftPI_bkup,tmps)
      |         set_param(gcb,'u16NShiftPI',tmps);
      |       end
      |     end
      |     if isnan(f32C1)
      |       if ~strcmp(f32C1_bkup,'0')
      |         set_param(gcb,'f32C1','0');
      |       end
      |     else
      |       tmps=num2str(f32C1);
      |       if ~strcmp(f32C1_bkup,tmps)
      |         set_param(gcb,'f32C1',tmps);
      |       end
      |     end
      |     if isnan(u16NShiftI)
      |       if ~strcmp(u16NShiftI_bkup,'0')
      |         set_param(gcb,'u16NShiftI','0');
      |       end
      |     else
      |       tmps=num2str(u16NShiftI);
      |       if ~strcmp(u16NShiftI_bkup,tmps)
      |         set_param(gcb,'u16NShiftI',tmps);
      |       end
      |     end
      |   else
      |     param=p.getParameter('uscale');
      |     if strcmp(param.Enabled,'on')
      |       hintText.Prompt='Caution: Implementation parameters are fixed.';
      |       p=Simulink.Mask.get(gcb);
      |       param=p.getParameter('if0');
      |       param.set('Enabled','off');
      |       param=p.getParameter('iksi');
      |       param.set('Enabled','off');
      |       param=p.getParameter('mechspeed');
      |       param.set('Enabled','off');
      |       param=p.getParameter('polepairs');
      |       param.set('Enabled','off');
      |       param=p.getParameter('ADCMaxError');
      |       param.set('Enabled','off');
      |       param=p.getParameter('uscale');
      |       param.set('Enabled','off');
      |     end
      |   end
      | end
      mask DialogControl CompBut Prompt: Recalculate sample times
      mask DialogControl CompBut Tooltip: Simulink updates the sample times of all blocks when the simulation is run. This button will update the sample times now.
      mask DialogControl CompBut Callback:
      | btn=questdlg('This will apply all changes in all open dialog boxes and update the schematic. Do you want to proceed?','Apply all changes','Continue','Cancel','Continue');
      | if strcmp(btn,'Continue')
      |   dlgs=DAStudio.ToolRoot.getOpenDialogs;
      |   for i=1:length(dlgs)
      |     dlgs(i).apply;
      |   end
      |   try
      |     SampleTime_1=str2double(get_param(gcb,'SampleTime_1'));
      |     ts=Simulink.Block.getSampleTimes(gcb);
      |     ts=ts(1).Value(1);
      |     if (SampleTime_1 ~= ts)
      |       SampleTime_1=ts;
      |       set_param(gcb,'SampleTime_1',num2str(ts));
      |       autoCalcEn=get_param(gcb,'autoCalcEn');
      |       if strcmp(autoCalcEn,'on')
      |         SampleTime=Simulink.data.evalinGlobal(bdroot,get_param(gcb,'SampleTime'));
      |         p=Simulink.Mask.get(gcb);
      |         hintText=p.getDialogControl('timeHint');
      |         if SampleTime==-1
      |           SampleTime=SampleTime_1;
      |           hintText.Prompt='Caution: Implementation parameters depend on inherited sample time. Make sure that the sample time of the block''s inputs corresponds to the sampling period in the target application.';
      |         else
      |           hintText.Prompt='Caution: Implementation parameters depend on the sample time. Make sure that the simulation time step corresponds to the sampling period in the target application.';
      |         end
      |         f32ADCMaxError_bkup=get_param(gcb,'f32ADCMaxError');
      |         f32CC1sc_bkup=get_param(gcb,'f32CC1sc');
      |         f32CC2sc_bkup=get_param(gcb,'f32CC2sc');
      |         f32UpperLimit_bkup=get_param(gcb,'f32UpperLimit');
      |         f32LowerLimit_bkup=get_param(gcb,'f32LowerLimit');
      |         u16NShiftPI_bkup=get_param(gcb,'u16NShiftPI');
      |         f32C1_bkup=get_param(gcb,'f32C1');
      |         u16NShiftI_bkup=get_param(gcb,'u16NShiftI');
      |         if0=Simulink.data.evalinGlobal(bdroot,get_param(gcb,'if0'));
      |         iksi=Simulink.data.evalinGlobal(bdroot,get_param(gcb,'iksi'));
      |         mechspeed=Simulink.data.evalinGlobal(bdroot,get_param(gcb,'mechspeed'));
      |         polepairs=Simulink.data.evalinGlobal(bdroot,get_param(gcb,'polepairs'));
      |         ADCMaxError=Simulink.data.evalinGlobal(bdroot,get_param(gcb,'ADCMaxError'));
      |         uscale=Simulink.data.evalinGlobal(bdroot,get_param(gcb,'uscale'));
      |         if (if0<=0)
      |           warning('Natural frequency f0 must be positive.');
      |         end
      |         if (iksi<=0)
      |           warning('Feedback loop attenuation must be positive.');
      |         end
      |         if (iksi>1)
      |           warning('Feedback loop attenuation must not exceed 1.');
      |         end
      |         if (mechspeed<=0)
      |           warning('Max. speed must be positive.');
      |         end
      |         if (polepairs<1)
      |           warning('Number of pole pairs must be a natural number (1, 2, 3, ...).');
      |         end
      |         if (round(polepairs)~=polepairs)
      |           warning('Number of pole pairs must be a natural number (1, 2, 3, ...).');
      |         end
      |         if (ADCMaxError<=0)
      |           warning('f32ADCMaxError must be positive.');
      |         end
      |         adcsc=ADCMaxError/uscale;
      |         f32ADCMaxError=round(adcsc*2^31);
      |         if f32ADCMaxError>2^31-1
      |           f32ADCMaxError=2^31-1;
      |           warning(['Parameter f32ADCMaxError of ' gcb ' exceeds the fixed-point range.']);
      |         end
      |         if f32ADCMaxError<-2^31
      |           f32ADCMaxError=-2^31;
      |           warning(['Parameter f32ADCMaxError of ' gcb ' exceeds the fixed-point range.']);
      |         end
      |         pgain=12.56637061435917*iksi*if0;
      |         igain=39.47841760435743*if0*if0;
      |         cc1=pgain+igain*SampleTime*0.5;
      |         cc2=-pgain+igain*SampleTime*0.5;
      |         wmax=polepairs*mechspeed*0.1047197551196598;
      |         cc1f=cc1*3.141592653589793/wmax;
      |         cc2f=cc2*3.141592653589793/wmax;
      |         u16NShiftPI=ceil(log2(abs(cc1f)));
      |         tmpsh=ceil(log2(abs(cc2f)));
      |         if u16NShiftPI<tmpsh
      |           u16NShiftPI=tmpsh;
      |         end
      |         if u16NShiftPI<0
      |           u16NShiftPI=0;
      |         end
      |         if u16NShiftPI>31
      |           u16NShiftPI=31;
      |           warning(['Parameter u16NShiftPI of ' gcb ' exceeds the fixed-point range.']);
      |         end
      |         f32CC1sc=round(cc1f*2^(-u16NShiftPI)*2^31);
      |         if f32CC1sc>2^31-1
      |           f32CC1sc=2^31-1;
      |           warning(['Parameter f32CC1sc of ' gcb ' exceeds the fixed-point range.']);
      |         end
      |         if f32CC1sc<-2^31
      |           f32CC1sc=-2^31;
      |           warning(['Parameter f32CC1sc of ' gcb ' exceeds the fixed-point range.']);
      |         end
      |         f32CC2sc=round(cc2f*2^(-u16NShiftPI)*2^31);
